simulink model "Test1_2"  (R2021a)
settings: Solver=FixedStepAuto  StartTime=0  StopTime=0.2  FixedStep=0.2  RelTol=1e-3
libraries: spsDistributedParametersLineLib x60, spsThreePhaseSeriesRLCLoadLib x20, spsThreePhaseVIMeasurementLib x4, spsGroundLib x1, spsThreePhaseSourceLib x1, spsSeriesRLCBranchLib x1, spspowerguiLib x1
settings Model: Creator=Admin  LastModifiedBy=Admin

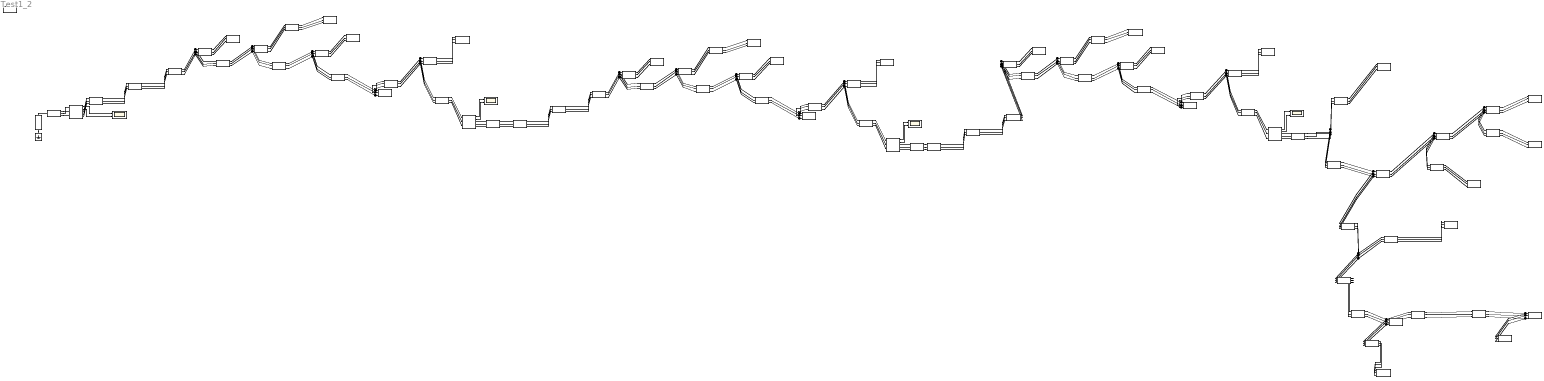
== system Test1_2 ==
  Ground : spsGroundLib/Ground  LConnTagsString=a
  Line 1 : spsDistributedParametersLineLib/Distributed Parameters Line  Phases=3  Length=0.24  Frequency=50  Resistance=[0.646656091154803 0.0486237908083191 0.0486712220507153;0.0486237908083191 0.646561225344642 0.0486237934466192;0.0486712220507153 0.0486237934466192 0.646656091154803]  Inductance=[0.00282448912315926 0.00133270803418135 0.00132951476746136;0.00133270803418135 0.00282479813276775 0.00133799988507366;0.00132951476746136 0.00133799988507366 0.00282448912315926]  Capacitance=[7.89543174552926e-09 -1.85986777702161e-09 -1.7901190036642e-09;-1.85986777702161e-09 7.82540023894543e-09 -1.8957321828871e-09;-1.7901190036642e-09 -1.8957321828871e-09 7.91264394645417e-09]  x1=[156.965405779652 1871.38054427965 1874.40865599682;314.159265358979 314.159265358979 314.159265358979;0.993745600560131 -0.794119316260784 -2.36332785011813]  x2=[156.969311652178 1871.26228409431 1874.29035744918;314.159265358979 314.159265358979 314.159265358979;0.993735016582748 -0.794173336848075 -2.36338159096693]  x3=[0.137596682921067 3.90971974679108 3.95295362832676;314.159265358979 314.159265358979 314.159265358979;0.924963946831068 -0.803256789057363 -2.37264678467375]  x4=[0.137502761428777 5.61255406681359 5.65797563637533;314.159265358979 314.159265358979 314.159265358979;1.0622023156878 -0.788043484537009 -2.35710686392184]  x5=1.14995345102668e-06  V1=ones(3,3)  V2=ones(3,3)  I1=ones(3,3)  I2=ones(3,3)  nHarmo=1  Measurements=None  Decoupling=off  VsMag0=0  VrMag0=0  VsAngle0=0  VrAngle0=0  IsMag0=0  IrMag0=0  IsAngle0=0  IrAngle0=0
      settings: SourceProductBaseCode=PS
  Line 10 : spsDistributedParametersLineLib/Distributed Parameters Line  Phases=3  Length=0.17001  Frequency=50  Resistance=[0.646656091154803 0.0486237908083191 0.0486712220507153;0.0486237908083191 0.646561225344642 0.0486237934466192;0.0486712220507153 0.0486237934466192 0.646656091154803]  Inductance=[0.00282448912315926 0.00133270803418135 0.00132951476746136;0.00133270803418135 0.00282479813276775 0.00133799988507366;0.00132951476746136 0.00133799988507366 0.00282448912315926]  Capacitance=[7.89543174552926e-09 -1.85986777702161e-09 -1.7901190036642e-09;-1.85986777702161e-09 7.82540023894543e-09 -1.8957321828871e-09;-1.7901190036642e-09 -1.8957321828871e-09 7.91264394645417e-09]  x1=[152.36017586446 2437.89117531741 2440.98179824564;314.159265358979 314.159265358979 314.159265358979;0.986975522658831 -0.641771871808401 -2.211874437678]  x2=[152.360654227211 2437.82903835373 2440.91967974814;314.159265358979 314.159265358979 314.159265358979;0.986975936673677 -0.641781263273401 -2.21188373356873]  x3=[0.133985232494409 5.71786094267282 5.77269147189891;314.159265358979 314.159265358979 314.159265358979;0.97714846741076 -0.614289076815549 -2.18464823198113]  x4=[0.132433471923299 6.69193998518046 6.74818842330152;314.159265358979 314.159265358979 314.159265358979;0.996660724368349 -0.66545069261843 -2.23536155506213]  x5=8.14598275871021e-07  V1=ones(3,3)  V2=ones(3,3)  I1=ones(3,3)  I2=ones(3,3)  nHarmo=1  Measurements=None  Decoupling=off  VsMag0=0  VrMag0=0  VsAngle0=0  VrAngle0=0  IsMag0=0  IrMag0=0  IsAngle0=0  IrAngle0=0
      settings: SourceProductBaseCode=PS
  Line 11 : spsDistributedParametersLineLib/Distributed Parameters Line  Phases=3  Length=0.27999  Frequency=50  Resistance=[0.646656091154803 0.0486237908083191 0.0486712220507153;0.0486237908083191 0.646561225344642 0.0486237934466192;0.0486712220507153 0.0486237934466192 0.646656091154803]  Inductance=[0.00282448912315926 0.00133270803418135 0.00132951476746136;0.00133270803418135 0.00282479813276775 0.00133799988507366;0.00132951476746136 0.00133799988507366 0.00282448912315926]  Capacitance=[7.89543174552926e-09 -1.85986777702161e-09 -1.7901190036642e-09;-1.85986777702161e-09 7.82540023894543e-09 -1.8957321828871e-09;-1.7901190036642e-09 -1.8957321828871e-09 7.91264394645417e-09]  x1=[149.797050896305 2771.33912653979 2774.29965117019;314.159265358979 314.159265358979 314.159265358979;0.982741259196518 -0.584603477585544 -2.15500920101434]  x2=[152.36017586446 2437.89117531741 2440.98179824564;314.159265358979 314.159265358979 314.159265358979;0.98680997135433 -0.641903391446747 -2.21200608251373]  x3=[5.10032716906624 1708.06752482602 1710.82869814989;314.159265358979 314.159265358979 314.159265358979;0.0770321916931183 2.28203627723541 0.713549765238094]  x4=[4.94208106497761 1720.91266597234 1723.79335570085;314.159265358979 314.159265358979 314.159265358979;-3.10669073601587 -0.857667050459027 -2.42615340559462]  x5=1.341564444804e-06  V1=ones(3,3)  V2=ones(3,3)  I1=ones(3,3)  I2=ones(3,3)  nHarmo=1  Measurements=None  Decoupling=off  VsMag0=0  VrMag0=0  VsAngle0=0  VrAngle0=0  IsMag0=0  IrMag0=0  IsAngle0=0  IrAngle0=0
      settings: SourceProductBaseCode=PS
  Line 12 : spsDistributedParametersLineLib/Distributed Parameters Line  Phases=3  Length=0.01  Frequency=50  Resistance=[0.646656091154803 0.0486237908083191 0.0486712220507153;0.0486237908083191 0.646561225344642 0.0486237934466192;0.0486712220507153 0.0486237934466192 0.646656091154803]  Inductance=[0.00282448912315926 0.00133270803418135 0.00132951476746136;0.00133270803418135 0.00282479813276775 0.00133799988507366;0.00132951476746136 0.00133799988507366 0.00282448912315926]  Capacitance=[7.89543174552926e-09 -1.85986777702161e-09 -1.7901190036642e-09;-1.85986777702161e-09 7.82540023894543e-09 -1.8957321828871e-09;-1.7901190036642e-09 -1.8957321828871e-09 7.91264394645417e-09]  x1=[149.705553633054 2783.39576802834 2786.35027775329;314.159265358979 314.159265358979 314.159265358979;0.982999779940424 -0.582489121625129 -2.15290363454968]  x2=[149.797050896305 2771.33912653979 2774.29965117019;314.159265358979 314.159265358979 314.159265358979;0.983147671241456 -0.584280609908175 -2.15468602598981]  x3=[5.10074508935649 1708.39159422601 1711.15572048992;314.159265358979 314.159265358979 314.159265358979;0.0774245703226859 2.28234705420157 0.713860837153466]  x4=[4.94342316518712 1721.99747040041 1724.88811393859;314.159265358979 314.159265358979 314.159265358979;-3.10585986858964 -0.857009678007319 -2.42549540948617]  x5=4.79147271261115e-08  V1=ones(3,3)  V2=ones(3,3)  I1=ones(3,3)  I2=ones(3,3)  nHarmo=1  Measurements=None  Decoupling=off  VsMag0=0  VrMag0=0  VsAngle0=0  VrAngle0=0  IsMag0=0  IrMag0=0  IsAngle0=0  IrAngle0=0
      settings: SourceProductBaseCode=PS
  Line 13 : spsDistributedParametersLineLib/Distributed Parameters Line  Phases=3  Length=0.04  Frequency=50  Resistance=[0.646656091154803 0.0486237908083191 0.0486712220507153;0.0486237908083191 0.646561225344642 0.0486237934466192;0.0486712220507153 0.0486237934466192 0.646656091154803]  Inductance=[0.00282448912315926 0.00133270803418135 0.00132951476746136;0.00133270803418135 0.00282479813276775 0.00133799988507366;0.00132951476746136 0.00133799988507366 0.00282448912315926]  Capacitance=[7.89543174552926e-09 -1.85986777702161e-09 -1.7901190036642e-09;-1.85986777702161e-09 7.82540023894543e-09 -1.8957321828871e-09;-1.7901190036642e-09 -1.8957321828871e-09 7.91264394645417e-09]  x1=[149.339597083059 2831.70975798566 2834.63941721022;314.159265358979 314.159265358979 314.159265358979;0.982361245048393 -0.575511762998782 -2.14596168775407]  x2=[149.705553633055 2783.39576802834 2786.35027775329;314.159265358979 314.159265358979 314.159265358979;0.982954621374002 -0.582524997140226 -2.15293954421573]  x3=[5.10056470112681 1708.24829976189 1711.01111492172;314.159265358979 314.159265358979 314.159265358979;0.0773196242206305 2.28226328792446 0.713776990731191]  x4=[4.94340800824378 1721.98418896766 1724.87470903959;314.159265358979 314.159265358979 314.159265358979;-3.10588973167749 -0.857033624646841 -2.42551937913716]  x5=1.91658908504446e-07  V1=ones(3,3)  V2=ones(3,3)  I1=ones(3,3)  I2=ones(3,3)  nHarmo=1  Measurements=None  Decoupling=off  VsMag0=0  VrMag0=0  VsAngle0=0  VrAngle0=0  IsMag0=0  IrMag0=0  IsAngle0=0  IrAngle0=0
      settings: SourceProductBaseCode=PS
  Line 14 : spsDistributedParametersLineLib/Distributed Parameters Line  Phases=3  Length=0.24001  Frequency=50  Resistance=[0.646656091154803 0.0486237908083191 0.0486712220507153;0.0486237908083191 0.646561225344642 0.0486237934466192;0.0486712220507153 0.0486237934466192 0.646656091154803]  Inductance=[0.00282448912315926 0.00133270803418135 0.00132951476746136;0.00133270803418135 0.00282479813276775 0.00133799988507366;0.00132951476746136 0.00133799988507366 0.00282448912315926]  Capacitance=[7.89543174552926e-09 -1.85986777702161e-09 -1.7901190036642e-09;-1.85986777702161e-09 7.82540023894543e-09 -1.8957321828871e-09;-1.7901190036642e-09 -1.8957321828871e-09 7.91264394645417e-09]  x1=[147.366559624798 3124.27831554393 3127.12738116645;314.159265358979 314.159265358979 314.159265358979;0.977740300651082 -0.53827513849313 -2.10890856037845]  x2=[149.339597082437 2831.70975810682 2834.63941733118;314.159265358979 314.159265358979 314.159265358979;0.982060172883721 -0.575750945040668 -2.14620109748057]  x3=[4.69597972482398 1707.56618859991 1710.7915439131;314.159265358979 314.159265358979 314.159265358979;0.150881701422709 2.28144587423602 0.712853079667161]  x4=[4.52474633855033 1722.028392532 1725.38783678718;314.159265358979 314.159265358979 314.159265358979;-3.03298242084286 -0.857513917481596 -2.42610561272272]  x5=1.1500013657538e-06  V1=ones(3,3)  V2=ones(3,3)  I1=ones(3,3)  I2=ones(3,3)  nHarmo=1  Measurements=None  Decoupling=off  VsMag0=0  VrMag0=0  VsAngle0=0  VrAngle0=0  IsMag0=0  IrMag0=0  IsAngle0=0  IrAngle0=0
      settings: SourceProductBaseCode=PS
  Line 15 : spsDistributedParametersLineLib/Distributed Parameters Line  Phases=3  Length=0.17  Frequency=50  Resistance=[0.646656091154803 0.0486237908083191 0.0486712220507153;0.0486237908083191 0.646561225344642 0.0486237934466192;0.0486712220507153 0.0486237934466192 0.646656091154803]  Inductance=[0.00282448912315926 0.00133270803418135 0.00132951476746136;0.00133270803418135 0.00282479813276775 0.00133799988507366;0.00132951476746136 0.00133799988507366 0.00282448912315926]  Capacitance=[7.89543174552926e-09 -1.85986777702161e-09 -1.7901190036642e-09;-1.85986777702161e-09 7.82540023894543e-09 -1.8957321828871e-09;-1.7901190036642e-09 -1.8957321828871e-09 7.91264394645417e-09]  x1=[132.899841984529 5355.36116411885 5357.02335058589;314.159265358979 314.159265358979 314.159265358979;0.942020039880082 -0.391447182887755 -1.96269694426104]  x2=[132.900799709299 5355.22518061845 5356.8875370799;314.159265358979 314.159265358979 314.159265358979;0.942023005810223 -0.391455476704388 -1.96270514529814]  x3=[0.118536716166914 12.5926352479183 12.7008603036067;314.159265358979 314.159265358979 314.159265358979;0.922749204209291 -0.36138822130875 -1.93290685330754]  x4=[0.113887175748437 14.6699901164864 14.7794661915918;314.159265358979 314.159265358979 314.159265358979;0.961819622301432 -0.417445208664834 -1.98849312716543]  x5=8.14550361143895e-07  V1=ones(3,3)  V2=ones(3,3)  I1=ones(3,3)  I2=ones(3,3)  nHarmo=1  Measurements=None  Decoupling=off  VsMag0=0  VrMag0=0  VsAngle0=0  VrAngle0=0  IsMag0=0  IrMag0=0  IsAngle0=0  IrAngle0=0
      settings: SourceProductBaseCode=PS
  Line 16 : spsDistributedParametersLineLib/Distributed Parameters Line  Phases=3  Length=0.27999  Frequency=50  Resistance=[0.646656091154803 0.0486237908083191 0.0486712220507153;0.0486237908083191 0.646561225344642 0.0486237934466192;0.0486712220507153 0.0486237934466192 0.646656091154803]  Inductance=[0.00282448912315926 0.00133270803418135 0.00132951476746136;0.00133270803418135 0.00282479813276775 0.00133799988507366;0.00132951476746136 0.00133799988507366 0.00282448912315926]  Capacitance=[7.89543174552926e-09 -1.85986777702161e-09 -1.7901190036642e-09;-1.85986777702161e-09 7.82540023894543e-09 -1.8957321828871e-09;-1.7901190036642e-09 -1.8957321828871e-09 7.91264394645417e-09]  x1=[130.625805916313 5714.43330932926 5715.86450257811;314.159265358979 314.159265358979 314.159265358979;0.935455723402759 -0.378911532038673 -1.9502060628031]  x2=[132.899841984529 5355.36116411885 5357.02335058588;314.159265358979 314.159265358979 314.159265358979;0.941854473522726 -0.391578714484606 -1.96282860106665]  x3=[4.69943627260133 1705.04689657621 1708.22372245339;314.159265358979 314.159265358979 314.159265358979;0.147579410474112 2.27912018503212 0.710521164983193]  x4=[4.54038793511918 1730.11014591192 1733.52103743161;314.159265358979 314.159265358979 314.159265358979;-3.03009591800017 -0.854995304416789 -2.42358856047792]  x5=1.341564444804e-06  V1=ones(3,3)  V2=ones(3,3)  I1=ones(3,3)  I2=ones(3,3)  nHarmo=1  Measurements=None  Decoupling=off  VsMag0=0  VrMag0=0  VsAngle0=0  VrAngle0=0  IsMag0=0  IrMag0=0  IsAngle0=0  IrAngle0=0
      settings: SourceProductBaseCode=PS
  Line 17 : spsDistributedParametersLineLib/Distributed Parameters Line  Phases=3  Length=0.01  Frequency=50  Resistance=[0.646656091154803 0.0486237908083191 0.0486712220507153;0.0486237908083191 0.646561225344642 0.0486237934466192;0.0486712220507153 0.0486237934466192 0.646656091154803]  Inductance=[0.00282448912315926 0.00133270803418135 0.00132951476746136;0.00133270803418135 0.00282479813276775 0.00133799988507366;0.00132951476746136 0.00133799988507366 0.00282448912315926]  Capacitance=[7.89543174552926e-09 -1.85986777702161e-09 -1.7901190036642e-09;-1.85986777702161e-09 7.82540023894543e-09 -1.8957321828871e-09;-1.7901190036642e-09 -1.8957321828871e-09 7.91264394645417e-09]  x1=[130.544687715025 5727.27361859197 5728.69645510391;314.159265358979 314.159265358979 314.159265358979;0.935629480507103 -0.378165636098579 -1.9494613242192]  x2=[130.625805916313 5714.43330932926 5715.86450257811;314.159265358979 314.159265358979 314.159265358979;0.935862135447697 -0.378588664361305 -1.94988288777856]  x3=[4.69982164193658 1705.36967379669 1708.54951574632;314.159265358979 314.159265358979 314.159265358979;0.147971637319338 2.2794306267218 0.710831898749288]  x4=[4.5416219595263 1731.19877594442 1734.619968649;314.159265358979 314.159265358979 314.159265358979;-3.0292654752636 -0.854338819679799 -2.42293145950432]  x5=4.79147271261115e-08  V1=ones(3,3)  V2=ones(3,3)  I1=ones(3,3)  I2=ones(3,3)  nHarmo=1  Measurements=None  Decoupling=off  VsMag0=0  VrMag0=0  VsAngle0=0  VrAngle0=0  IsMag0=0  IrMag0=0  IsAngle0=0  IrAngle0=0
      settings: SourceProductBaseCode=PS
  Line 18 : spsDistributedParametersLineLib/Distributed Parameters Line  Phases=3  Length=0.04  Frequency=50  Resistance=[0.646656091154803 0.0486237908083191 0.0486712220507153;0.0486237908083191 0.646561225344642 0.0486237934466192;0.0486712220507153 0.0486237934466192 0.646656091154803]  Inductance=[0.00282448912315926 0.00133270803418135 0.00132951476746136;0.00133270803418135 0.00282479813276775 0.00133799988507366;0.00132951476746136 0.00133799988507366 0.00282448912315926]  Capacitance=[7.89543174552926e-09 -1.85986777702161e-09 -1.7901190036642e-09;-1.85986777702161e-09 7.82540023894543e-09 -1.8957321828871e-09;-1.7901190036642e-09 -1.8957321828871e-09 7.91264394645417e-09]  x1=[130.220285493845 5778.64498268911 5780.03432477456;314.159265358979 314.159265358979 314.159265358979;0.934650804974626 -0.376528198600221 -1.94782969786199]  x2=[130.544687715024 5727.27361859198 5728.69645510391;314.159265358979 314.159265358979 314.159265358979;0.935584321940681 -0.378201511613676 -1.94949723388525]  x3=[4.69965556978429 1705.22633120538 1708.40482377799;314.159265358979 314.159265358979 314.159265358979;0.1478666288771 2.27934671978969 0.710747910420055]  x4=[4.54160812738084 1731.18526113571 1734.60632300578;314.159265358979 314.159265358979 314.159265358979;-3.02929537261956 -0.854362839392123 -2.4229555028762]  x5=1.91658908504446e-07  V1=ones(3,3)  V2=ones(3,3)  I1=ones(3,3)  I2=ones(3,3)  nHarmo=1  Measurements=None  Decoupling=off  VsMag0=0  VrMag0=0  VsAngle0=0  VrAngle0=0  IsMag0=0  IrMag0=0  IsAngle0=0  IrAngle0=0
      settings: SourceProductBaseCode=PS
  Line 19 : spsDistributedParametersLineLib/Distributed Parameters Line  Phases=3  Length=0.02  Frequency=50  Resistance=[0.646656091154803 0.0486237908083191 0.0486712220507153;0.0486237908083191 0.646561225344642 0.0486237934466192;0.0486712220507153 0.0486237934466192 0.646656091154803]  Inductance=[0.00282448912315926 0.00133270803418135 0.00132951476746136;0.00133270803418135 0.00282479813276775 0.00133799988507366;0.00132951476746136 0.00133799988507366 0.00282448912315926]  Capacitance=[7.89543174552926e-09 -1.85986777702161e-09 -1.7901190036642e-09;-1.85986777702161e-09 7.82540023894543e-09 -1.8957321828871e-09;-1.7901190036642e-09 -1.8957321828871e-09 7.91264394645417e-09]  x1=[147.366559624798 3124.27831554393 3127.12738116645;314.159265358979 314.159265358979 314.159265358979;0.978071478524361 -0.538012039423913 -2.10864521085755]  x2=[147.366576589391 3124.27609299989 3127.1251586601;314.159265358979 314.159265358979 314.159265358979;0.978071529284701 -0.538012448077892 -2.10864561647098]  x3=[0.129209254301903 7.78403106502851 7.85222208431091;314.159265358979 314.159265358979 314.159265358979;0.975452703470751 -0.534902174377798 -2.10556665489213]  x4=[0.128484600405194 8.11756536104211 8.18611566687072;314.159265358979 314.159265358979 314.159265358979;0.980674883603026 -0.5410179521277 -2.11162204802365]  x5=9.5829454252223e-08  V1=ones(3,3)  V2=ones(3,3)  I1=ones(3,3)  I2=ones(3,3)  nHarmo=1  Measurements=None  Decoupling=off  VsMag0=0  VrMag0=0  VsAngle0=0  VrAngle0=0  IsMag0=0  IrMag0=0  IsAngle0=0  IrAngle0=0
      settings: SourceProductBaseCode=PS
  Line 2 : spsDistributedParametersLineLib/Distributed Parameters Line  Phases=3  Length=0.02  Frequency=50  Resistance=[0.646656091154803 0.0486237908083191 0.0486712220507153;0.0486237908083191 0.646561225344642 0.0486237934466192;0.0486712220507153 0.0486237934466192 0.646656091154803]  Inductance=[0.00282448912315926 0.00133270803418135 0.00132951476746136;0.00133270803418135 0.00282479813276775 0.00133799988507366;0.00132951476746136 0.00133799988507366 0.00282448912315926]  Capacitance=[7.89543174552926e-09 -1.85986777702161e-09 -1.7901190036642e-09;-1.85986777702161e-09 7.82540023894543e-09 -1.8957321828871e-09;-1.7901190036642e-09 -1.8957321828871e-09 7.91264394645417e-09]  x1=[156.965405779652 1871.38054427965 1874.40865599682;314.159265358979 314.159265358979 314.159265358979;0.994076763380555 -0.793856229150073 -2.36306451256712]  x2=[156.965417517027 1871.37888626964 1874.40699915953;314.159265358979 314.159265358979 314.159265358979;0.994076744009357 -0.793856337139222 -2.3630646177889]  x3=[0.137288875738453 4.66877336660217 4.71294070353627;314.159265358979 314.159265358979 314.159265358979;0.991734266986629 -0.781676589050808 -2.3509868412552]  x4=[0.137189890045939 4.85660166120808 4.9011132957881;314.159265358979 314.159265358979 314.159265358979;0.996390813875115 -0.805588362177722 -2.3747020378792]  x5=9.5829454252223e-08  V1=ones(3,3)  V2=ones(3,3)  I1=ones(3,3)  I2=ones(3,3)  nHarmo=1  Measurements=None  Decoupling=off  VsMag0=0  VrMag0=0  VsAngle0=0  VrAngle0=0  IsMag0=0  IrMag0=0  IsAngle0=0  IrAngle0=0
      settings: SourceProductBaseCode=PS
  Line 20 : spsDistributedParametersLineLib/Distributed Parameters Line  Phases=3  Length=0.5  Frequency=50  Resistance=[0.646656091154803 0.0486237908083191 0.0486712220507153;0.0486237908083191 0.646561225344642 0.0486237934466192;0.0486712220507153 0.0486237934466192 0.646656091154803]  Inductance=[0.00282448912315926 0.00133270803418135 0.00132951476746136;0.00133270803418135 0.00282479813276775 0.00133799988507366;0.00132951476746136 0.00133799988507366 0.00282448912315926]  Capacitance=[7.89543174552926e-09 -1.85986777702161e-09 -1.7901190036642e-09;-1.85986777702161e-09 7.82540023894543e-09 -1.8957321828871e-09;-1.7901190036642e-09 -1.8957321828871e-09 7.91264394645417e-09]  x1=[143.264957244536 3744.49816369777 3747.08832907544;314.159265358979 314.159265358979 314.159265358979;0.967966773621725 -0.479516643242202 -2.05041928603723]  x2=[147.366559624798 3124.27831554393 3127.12738116645;314.159265358979 314.159265358979 314.159265358979;0.977348941461618 -0.538586047665466 -2.1092197655143]  x3=[4.69457824125427 1706.09065502595 1709.30076063797;314.159265358979 314.159265358979 314.159265358979;0.149751318444868 2.28055339272289 0.71195954517954]  x4=[4.52557826260862 1722.47910674114 1725.84144140248;314.159265358979 314.159265358979 314.159265358979;-3.03299533225323 -0.85752144723027 -2.42611334880867]  x5=2.39573635630557e-06  V1=ones(3,3)  V2=ones(3,3)  I1=ones(3,3)  I2=ones(3,3)  nHarmo=1  Measurements=None  Decoupling=off  VsMag0=0  VrMag0=0  VsAngle0=0  VrAngle0=0  IsMag0=0  IrMag0=0  IsAngle0=0  IrAngle0=0
      settings: SourceProductBaseCode=PS
  Line 21 : spsDistributedParametersLineLib/Distributed Parameters Line  Phases=3  Length=0.23  Frequency=50  Resistance=[0.646656091154803 0.0486237908083191 0.0486712220507153;0.0486237908083191 0.646561225344642 0.0486237934466192;0.0486712220507153 0.0486237934466192 0.646656091154803]  Inductance=[0.00282448912315926 0.00133270803418135 0.00132951476746136;0.00133270803418135 0.00282479813276775 0.00133799988507366;0.00132951476746136 0.00133799988507366 0.00282448912315926]  Capacitance=[7.89543174552926e-09 -1.85986777702161e-09 -1.7901190036642e-09;-1.85986777702161e-09 7.82540023894543e-09 -1.8957321828871e-09;-1.7901190036642e-09 -1.8957321828871e-09 7.91264394645417e-09]  x1=[141.381540716079 4033.34520134928 4035.78863035435;314.159265358979 314.159265358979 314.159265358979;0.963872150999868 -0.458142281050839 -2.02913402389008]  x2=[143.264957244536 3744.49816369777 3747.08832907544;314.159265358979 314.159265358979 314.159265358979;0.968373200719517 -0.479193763606329 -2.05009609904281]  x3=[4.69693280636161 1706.73403429122 1709.94265597579;314.159265358979 314.159265358979 314.159265358979;0.149813372942936 2.28064855389235 0.712053657755716]  x4=[4.53009342094595 1725.03316244308 1728.41207132862;314.159265358979 314.159265358979 314.159265358979;-3.03180886302381 -0.856556207454851 -2.42514832021994]  x5=1.10203872390056e-06  V1=ones(3,3)  V2=ones(3,3)  I1=ones(3,3)  I2=ones(3,3)  nHarmo=1  Measurements=None  Decoupling=off  VsMag0=0  VrMag0=0  VsAngle0=0  VrAngle0=0  IsMag0=0  IrMag0=0  IsAngle0=0  IrAngle0=0
      settings: SourceProductBaseCode=PS
  Line 22 : spsDistributedParametersLineLib/Distributed Parameters Line  Phases=3  Length=1.62  Frequency=50  Resistance=[0.80718830189013 0.0486237908083191 0.0486712220507153;0.0486237908083191 0.807093436079969 0.0486237934466192;0.0486712220507153 0.0486237934466192 0.80718830189013]  Inductance=[0.00279786707424938 0.00133270803418135 0.00132951476746136;0.00133270803418135 0.00279817608385787 0.00133799988507366;0.00132951476746136 0.00133799988507366 0.00279786707424938]  Capacitance=[7.73340098830622e-09 -1.79942827973291e-09 -1.73218055098733e-09;-1.79942827973291e-09 7.66505189233746e-09 -1.83375898618858e-09;-1.73218055098733e-09 -1.83375898618858e-09 7.749673531177e-09]  x1=[111.255817895821 4033.38117611576 4036.11238880674;314.159265358979 314.159265358979 314.159265358979;1.03593595279213 -0.464052863724388 -2.03502879066849]  x2=[111.256284671676 4033.37738573713 4036.10862101927;314.159265358979 314.159265358979 314.159265358979;1.03593486115945 -0.464056537743729 -2.03503248077632]  x3=[0.0968983486960544 10.2070175470074 10.2916609188853;314.159265358979 314.159265358979 314.159265358979;1.03318306869383 -0.465730267618516 -2.03670968562963]  x4=[0.0968282868719981 10.2221861600155 10.3068418342109;314.159265358979 314.159265358979 314.159265358979;1.03626767416038 -0.464279740581859 -2.03525380445823]  x5=7.70442045759223e-06  V1=ones(3,3)  V2=ones(3,3)  I1=ones(3,3)  I2=ones(3,3)  nHarmo=1  Measurements=None  Decoupling=off  VsMag0=0  VrMag0=0  VsAngle0=0  VrAngle0=0  IsMag0=0  IrMag0=0  IsAngle0=0  IrAngle0=0
      settings: SourceProductBaseCode=PS
  Line 23 : spsDistributedParametersLineLib/Distributed Parameters Line  Phases=3  Length=0.54002  Frequency=50  Resistance=[0.646656091154803 0.0486237908083191 0.0486712220507153;0.0486237908083191 0.646561225344642 0.0486237934466192;0.0486712220507153 0.0486237934466192 0.646656091154803]  Inductance=[0.00282448912315926 0.00133270803418135 0.00132951476746136;0.00133270803418135 0.00282479813276775 0.00133799988507366;0.00132951476746136 0.00133799988507366 0.00282448912315926]  Capacitance=[7.89543174552926e-09 -1.85986777702161e-09 -1.7901190036642e-09;-1.85986777702161e-09 7.82540023894543e-09 -1.8957321828871e-09;-1.7901190036642e-09 -1.8957321828871e-09 7.91264394645417e-09]  x1=[136.970854809158 4717.10989026672 4719.16622621704;314.159265358979 314.159265358979 314.159265358979;0.952352588146702 -0.419268144212771 -1.99041696083254]  x2=[141.381540716079 4033.34520134928 4035.78863035435;314.159265358979 314.159265358979 314.159265358979;0.963405482374469 -0.458513018623851 -2.02950511437901]  x3=[4.6950771769482 1704.92349425677 1708.11503821512;314.159265358979 314.159265358979 314.159265358979;0.1484970320043 2.2796412280549 0.711045424706869]  x4=[4.53057574604281 1725.22598750204 1728.60666973103;314.159265358979 314.159265358979 314.159265358979;-3.03196710314176 -0.856642086949454 -2.42523422570912]  x5=2.58749109426427e-06  V1=ones(3,3)  V2=ones(3,3)  I1=ones(3,3)  I2=ones(3,3)  nHarmo=1  Measurements=None  Decoupling=off  VsMag0=0  VrMag0=0  VsAngle0=0  VrAngle0=0  IsMag0=0  IrMag0=0  IsAngle0=0  IrAngle0=0
      settings: SourceProductBaseCode=PS
  Line 24 : spsDistributedParametersLineLib/Distributed Parameters Line  Phases=3  Length=0.13998  Frequency=50  Resistance=[0.646656091154803 0.0486237908083191 0.0486712220507153;0.0486237908083191 0.646561225344642 0.0486237934466192;0.0486712220507153 0.0486237934466192 0.646656091154803]  Inductance=[0.00282448912315926 0.00133270803418135 0.00132951476746136;0.00133270803418135 0.00282479813276775 0.00133799988507366;0.00132951476746136 0.00133799988507366 0.00282448912315926]  Capacitance=[7.89543174552926e-09 -1.85986777702161e-09 -1.7901190036642e-09;-1.85986777702161e-09 7.82540023894543e-09 -1.8957321828871e-09;-1.7901190036642e-09 -1.8957321828871e-09 7.91264394645417e-09]  x1=[136.970854809158 4717.10989026672 4719.16622621704;314.159265358979 314.159265358979 314.159265358979;0.952954762577076 -0.418789756177456 -1.98993811740569]  x2=[136.971666154249 4717.03540311946 4719.09183073719;314.159265358979 314.159265358979 314.159265358979;0.952955500131483 -0.418794373833103 -1.98994267847764]  x3=[0.121357845438818 11.3292840292329 11.4262147740208;314.159265358979 314.159265358979 314.159265358979;0.930714707543745 -0.394910744474516 -1.96626658224448]  x4=[0.118203608434895 12.6819047773621 12.7798105880992;314.159265358979 314.159265358979 314.159265358979;0.975575610247598 -0.440284325346567 -2.01126504900171]  x5=6.70710350311308e-07  V1=ones(3,3)  V2=ones(3,3)  I1=ones(3,3)  I2=ones(3,3)  nHarmo=1  Measurements=None  Decoupling=off  VsMag0=0  VrMag0=0  VsAngle0=0  VrAngle0=0  IsMag0=0  IrMag0=0  IsAngle0=0  IrAngle0=0
      settings: SourceProductBaseCode=PS
  Line 25 : spsDistributedParametersLineLib/Distributed Parameters Line  Phases=3  Length=0.14997  Frequency=50  Resistance=[0.476003738225748 0.351747138225748 0.351747138225748;0.351747138225748 0.476003738225748 0.351747138225748;0.351747138225748 0.351747138225748 0.476003738225748]  Inductance=[0.000705954362986426 0.000459934243504405 0.000459934243504405;0.000459934243504405 0.000705954362986426 0.000459934243504405;0.000459934243504405 0.000459934243504405 0.000705954362986426]  Capacitance=[5.7561313269996e-07 -1.37543883484145e-07 -1.37543912800485e-07;-1.37543883484145e-07 5.75613027339387e-07 -1.37543875208088e-07;-1.37543912800485e-07 -1.37543875208088e-07 5.75613005057695e-07]  x1=[77.3212987177548 4717.59725972927 4719.75403690061;314.159265358979 314.159265358979 314.159265358979;1.09142381613903 -0.337596063619059 -1.90863201691887]  x2=[77.3213406496756 4717.58057530735 4719.73734485071;314.159265358979 314.159265358979 314.159265358979;1.09142256389172 -0.337596336996628 -1.90863229029648]  x3=[1.04934913172663 253.129562662736 253.245268059759;314.159265358979 314.159265358979 314.159265358979;1.09038177152188 -0.336520492000803 -1.9075564451716]  x4=[1.04934910448407 254.481417052228 254.59774051285;314.159265358979 314.159265358979 314.159265358979;1.09142254929381 -0.339288761111601 -1.91032471449075]  x5=3.31498451375949e-06  V1=ones(3,3)  V2=ones(3,3)  I1=ones(3,3)  I2=ones(3,3)  nHarmo=1  Measurements=None  Decoupling=off  VsMag0=0  VrMag0=0  VsAngle0=0  VrAngle0=0  IsMag0=0  IrMag0=0  IsAngle0=0  IrAngle0=0
      settings: SourceProductBaseCode=PS
  Line 26 : spsDistributedParametersLineLib/Distributed Parameters Line  Phases=3  Length=0.50001  Frequency=50  Resistance=[0.646656091154803 0.0486237908083191 0.0486712220507153;0.0486237908083191 0.646561225344642 0.0486237934466192;0.0486712220507153 0.0486237934466192 0.646656091154803]  Inductance=[0.00282448912315926 0.00133270803418135 0.00132951476746136;0.00133270803418135 0.00282479813276775 0.00133799988507366;0.00132951476746136 0.00133799988507366 0.00282448912315926]  Capacitance=[7.89543174552926e-09 -1.85986777702161e-09 -1.7901190036642e-09;-1.85986777702161e-09 7.82540023894543e-09 -1.8957321828871e-09;-1.7901190036642e-09 -1.8957321828871e-09 7.91264394645417e-09]  x1=[132.899841984529 5355.36116411885 5357.02335058589;314.159265358979 314.159265358979 314.159265358979;0.941523280596591 -0.391841825512328 -1.96309196255744]  x2=[136.970854809158 4717.10989026672 4719.16622621704;314.159265358979 314.159265358979 314.159265358979;0.952412814621452 -0.419220298234136 -1.99036906930793]  x3=[4.69667848159883 1704.39660768418 1707.57684651848;314.159265358979 314.159265358979 314.159265358979;0.147653797922356 2.27911528105476 0.710517948064024]  x4=[4.53531416160052 1727.41542933722 1730.81042696937;314.159265358979 314.159265358979 314.159265358979;-3.0312239923196 -0.855926939645363 -2.42451941049668]  x5=2.3957842710327e-06  V1=ones(3,3)  V2=ones(3,3)  I1=ones(3,3)  I2=ones(3,3)  nHarmo=1  Measurements=None  Decoupling=off  VsMag0=0  VrMag0=0  VsAngle0=0  VrAngle0=0  IsMag0=0  IrMag0=0  IsAngle0=0  IrAngle0=0
      settings: SourceProductBaseCode=PS
  Line 3 : spsDistributedParametersLineLib/Distributed Parameters Line  Phases=3  Length=0.5  Frequency=50  Resistance=[0.646656091154803 0.0486237908083191 0.0486712220507153;0.0486237908083191 0.646561225344642 0.0486237934466192;0.0486712220507153 0.0486237934466192 0.646656091154803]  Inductance=[0.00282448912315926 0.00133270803418135 0.00132951476746136;0.00133270803418135 0.00282479813276775 0.00133799988507366;0.00132951476746136 0.00133799988507366 0.00282448912315926]  Capacitance=[7.89543174552926e-09 -1.85986777702161e-09 -1.7901190036642e-09;-1.85986777702161e-09 7.82540023894543e-09 -1.8957321828871e-09;-1.7901190036642e-09 -1.8957321828871e-09 7.91264394645417e-09]  x1=[156.956907595247 1871.66787959428 1874.69603995596;314.159265358979 314.159265358979 314.159265358979;0.993376948009191 -0.794314673924448 -2.36352415263414]  x2=[156.965405779652 1871.38054427965 1874.40865599682;314.159265358979 314.159265358979 314.159265358979;0.993354226317812 -0.794430237391626 -2.36363906722387]  x3=[0.137650868781888 3.81520206109773 3.85823350187218;314.159265358979 314.159265358979 314.159265358979;0.92153433973683 -0.789495270500456 -2.35903959755234]  x4=[0.137458609404139 5.70509774441842 5.7506581745733;314.159265358979 314.159265358979 314.159265358979;1.06454424282906 -0.798132971601806 -2.36712903812269]  x5=2.39573635630557e-06  V1=ones(3,3)  V2=ones(3,3)  I1=ones(3,3)  I2=ones(3,3)  nHarmo=1  Measurements=None  Decoupling=off  VsMag0=0  VrMag0=0  VsAngle0=0  VrAngle0=0  IsMag0=0  IrMag0=0  IsAngle0=0  IrAngle0=0
      settings: SourceProductBaseCode=PS
  Line 4 : spsDistributedParametersLineLib/Distributed Parameters Line  Phases=3  Length=0.23  Frequency=50  Resistance=[0.646656091154803 0.0486237908083191 0.0486712220507153;0.0486237908083191 0.646561225344642 0.0486237934466192;0.0486712220507153 0.0486237934466192 0.646656091154803]  Inductance=[0.00282448912315926 0.00133270803418135 0.00132951476746136;0.00133270803418135 0.00282479813276775 0.00133799988507366;0.00132951476746136 0.00133799988507366 0.00282448912315926]  Capacitance=[7.89543174552926e-09 -1.85986777702161e-09 -1.7901190036642e-09;-1.85986777702161e-09 7.82540023894543e-09 -1.8957321828871e-09;-1.7901190036642e-09 -1.8957321828871e-09 7.91264394645417e-09]  x1=[156.952553131653 1871.85294613081 1874.88113522112;314.159265358979 314.159265358979 314.159265358979;0.993793842090127 -0.79392653725406 -2.36313611703891]  x2=[156.956907595247 1871.66787959428 1874.69603995596;314.159265358979 314.159265358979 314.159265358979;0.993783375106984 -0.793991794288575 -2.36320096563972]  x3=[0.138137241015989 3.5006914421516 3.54316106458494;314.159265358979 314.159265358979 314.159265358979;0.915502409980736 -0.764168070499261 -2.33403697280712]  x4=[0.137139558374005 6.02613644564006 6.07225205821398;314.159265358979 314.159265358979 314.159265358979;1.07229801814102 -0.811481059773425 -2.3803832041032]  x5=1.10203872390056e-06  V1=ones(3,3)  V2=ones(3,3)  I1=ones(3,3)  I2=ones(3,3)  nHarmo=1  Measurements=None  Decoupling=off  VsMag0=0  VrMag0=0  VsAngle0=0  VrAngle0=0  IsMag0=0  IrMag0=0  IsAngle0=0  IrAngle0=0
      settings: SourceProductBaseCode=PS
  Line 44 : spsDistributedParametersLineLib/Distributed Parameters Line  Phases=3  Length=1.11  Frequency=50  Resistance=[0.502970710632245 0.0486237908083191 0.0486712220507153;0.0486237908083191 0.502875844822084 0.0486237934466192;0.0486712220507153 0.0486237934466192 0.502970710632245]  Inductance=[0.00286900545038753 0.00133270803418135 0.00132951476746136;0.00133270803418135 0.00286931445999602 0.00133799988507366;0.00132951476746136 0.00133799988507366 0.00286900545038753]  Capacitance=[8.11484299003193e-09 -1.94249816214699e-09 -1.86930692621136e-09;-1.94249816214699e-09 8.0425699231653e-09 -1.98049571960044e-09;-1.86930692621136e-09 -1.98049571960044e-09 8.13337738722527e-09]  x1=[173.362030490119 1870.46864326983 1872.93675817124;314.159265358979 314.159265358979 314.159265358979;0.925429746096986 -0.789510342867653 -2.35873222576214]  x2=[173.362277666248 1870.47039245228 1872.93851360611;314.159265358979 314.159265358979 314.159265358979;0.925429253884466 -0.789511220669717 -2.35873311112546]  x3=[0.151985260585037 4.75806840684685 4.80092870626659;314.159265358979 314.159265358979 314.159265358979;0.923740844335302 -0.790878375878761 -2.36010180165187]  x4=[0.151985260870719 4.75806840784355 4.80092870785854;314.159265358979 314.159265358979 314.159265358979;0.92542925320876 -0.789511220650776 -2.35873311108327]  x5=5.37516004033389e-06  V1=ones(3,3)  V2=ones(3,3)  I1=ones(3,3)  I2=ones(3,3)  nHarmo=1  Measurements=None  Decoupling=off  VsMag0=0  VrMag0=0  VsAngle0=0  VrAngle0=0  IsMag0=0  IrMag0=0  IsAngle0=0  IrAngle0=0
      settings: SourceProductBaseCode=PS
  Line 45 : spsDistributedParametersLineLib/Distributed Parameters Line  Phases=3  Length=0.03  Frequency=50  Resistance=[0.476003738225748 0.351747138225748 0.351747138225748;0.351747138225748 0.476003738225748 0.351747138225748;0.351747138225748 0.351747138225748 0.476003738225748]  Inductance=[0.000705954362986426 0.000459934243504405 0.000459934243504405;0.000459934243504405 0.000705954362986426 0.000459934243504405;0.000459934243504405 0.000459934243504405 0.000705954362986426]  Capacitance=[5.7561313269996e-07 -1.37543883484145e-07 -1.37543912800485e-07;-1.37543883484145e-07 5.75613027339387e-07 -1.37543875208088e-07;-1.37543912800485e-07 -1.37543875208088e-07 5.75613005057695e-07]  x1=[137.574489867811 1870.43821958496 1873.77265383368;314.159265358979 314.159265358979 314.159265358979;1.0926378669217 -0.712734679174021 -2.28197946476194]  x2=[137.574495166611 1870.43824928999 1873.77268368076;314.159265358979 314.159265358979 314.159265358979;1.09263774985956 -0.712734704669924 -2.2819794903938]  x3=[1.86971697622916 100.689759042347 100.869237693452;314.159265358979 314.159265358979 314.159265358979;1.09229955538654 -0.712924192925255 -2.28216957326277]  x4=[1.86979666932282 100.689742781977 100.869248230241;314.159265358979 314.159265358979 314.159265358979;1.09276769806716 -0.712670035796461 -2.28191422679785]  x5=6.63129528657629e-07  V1=ones(3,3)  V2=ones(3,3)  I1=ones(3,3)  I2=ones(3,3)  nHarmo=1  Measurements=None  Decoupling=off  VsMag0=0  VrMag0=0  VsAngle0=0  VrAngle0=0  IsMag0=0  IrMag0=0  IsAngle0=0  IrAngle0=0
      settings: SourceProductBaseCode=PS
  Line 46 : spsDistributedParametersLineLib/Distributed Parameters Line  Phases=3  Length=0.28003  Frequency=50  Resistance=[0.476003738225748 0.351747138225748 0.351747138225748;0.351747138225748 0.476003738225748 0.351747138225748;0.351747138225748 0.351747138225748 0.476003738225748]  Inductance=[0.000705954362986426 0.000459934243504405 0.000459934243504405;0.000459934243504405 0.000705954362986426 0.000459934243504405;0.000459934243504405 0.000459934243504405 0.000705954362986426]  Capacitance=[5.7561313269996e-07 -1.37543883484145e-07 -1.37543912800485e-07;-1.37543883484145e-07 5.75613027339387e-07 -1.37543875208088e-07;-1.37543912800485e-07 -1.37543875208088e-07 5.75613005057695e-07]  x1=[137.574489867811 1870.43821958496 1873.77265383368;314.159265358979 314.159265358979 314.159265358979;1.09090158954707 -0.713775125979268 -2.28301991148676]  x2=[137.574766367975 1870.43959233676 1873.77402962741;314.159265358979 314.159265358979 314.159265358979;1.09089676298152 -0.713776305655424 -2.2830210920491]  x3=[1.86411948827272 100.563600594904 100.74285874572;314.159265358979 314.159265358979 314.159265358979;1.08885867167533 -0.71498806739371 -2.28423327026689]  x4=[1.86417554032863 100.563589510719 100.742865766276;314.159265358979 314.159265358979 314.159265358979;1.0909928599777 -0.713729195375815 -2.2829735644268]  x5=6.18987206366653e-06  V1=ones(3,3)  V2=ones(3,3)  I1=ones(3,3)  I2=ones(3,3)  nHarmo=1  Measurements=None  Decoupling=off  VsMag0=0  VrMag0=0  VsAngle0=0  VrAngle0=0  IsMag0=0  IrMag0=0  IsAngle0=0  IrAngle0=0
      settings: SourceProductBaseCode=PS
  Line 47 : spsDistributedParametersLineLib/Distributed Parameters Line  Phases=3  Length=0.28003  Frequency=50  Resistance=[0.646656091154803 0.0486237908083191 0.0486712220507153;0.0486237908083191 0.646561225344642 0.0486237934466192;0.0486712220507153 0.0486237934466192 0.646656091154803]  Inductance=[0.00282448912315926 0.00133270803418135 0.00132951476746136;0.00133270803418135 0.00282479813276775 0.00133799988507366;0.00132951476746136 0.00133799988507366 0.00282448912315926]  Capacitance=[7.89543174552926e-09 -1.85986777702161e-09 -1.7901190036642e-09;-1.85986777702161e-09 7.82540023894543e-09 -1.8957321828871e-09;-1.7901190036642e-09 -1.8957321828871e-09 7.91264394645417e-09]  x1=[157.003522435008 1870.42653910552 1873.45371016496;314.159265358979 314.159265358979 314.159265358979;0.993627239752327 -0.794601201094145 -2.36380739557115]  x2=[157.003591771387 1870.42705832321 1873.45423118083;314.159265358979 314.159265358979 314.159265358979;0.993627050481464 -0.794601554289817 -2.36380775171645]  x3=[0.137255387038702 4.75851172908053 4.80280889948096;314.159265358979 314.159265358979 314.159265358979;0.992369761746573 -0.795597707622521 -2.36480477578221]  x4=[0.137254739530375 4.75851184516489 4.80280883918688;314.159265358979 314.159265358979 314.159265358979;0.994462989164056 -0.793939957467913 -2.36314560025828]  x5=1.3417561037125e-06  V1=ones(3,3)  V2=ones(3,3)  I1=ones(3,3)  I2=ones(3,3)  nHarmo=1  Measurements=None  Decoupling=off  VsMag0=0  VrMag0=0  VsAngle0=0  VrAngle0=0  IsMag0=0  IrMag0=0  IsAngle0=0  IrAngle0=0
      settings: SourceProductBaseCode=PS
  Line 48 : spsDistributedParametersLineLib/Distributed Parameters Line  Phases=3  Length=0.3  Frequency=50  Resistance=[0.80718830189013 0.0486237908083191 0.0486712220507153;0.0486237908083191 0.807093436079969 0.0486237934466192;0.0486712220507153 0.0486237934466192 0.80718830189013]  Inductance=[0.00279786707424938 0.00133270803418135 0.00132951476746136;0.00133270803418135 0.00279817608385787 0.00133799988507366;0.00132951476746136 0.00133799988507366 0.00279786707424938]  Capacitance=[7.73340098830622e-09 -1.79942827973291e-09 -1.73218055098733e-09;-1.79942827973291e-09 7.66505189233746e-09 -1.83375898618858e-09;-1.73218055098733e-09 -1.83375898618858e-09 7.749673531177e-09]  x1=[145.468327536726 1870.40466979634 1873.84374807451;314.159265358979 314.159265358979 314.159265358979;1.05282340055429 -0.798852585888835 -2.36802347632596]  x2=[145.468342149325 1870.40478533662 1873.84386402286;314.159265358979 314.159265358979 314.159265358979;1.05282334763226 -0.798852687387431 -2.36802357866973]  x3=[0.126748186136066 4.74586358195713 4.7908156688179;314.159265358979 314.159265358979 314.159265358979;1.05237514924046 -0.799204127438348 -2.36837531514946]  x4=[0.126748186850792 4.74586358220615 4.79081566884878;314.159265358979 314.159265358979 314.159265358979;1.05282334746568 -0.798852687304644 -2.36802357870356]  x5=1.42674452918375e-06  V1=ones(3,3)  V2=ones(3,3)  I1=ones(3,3)  I2=ones(3,3)  nHarmo=1  Measurements=None  Decoupling=off  VsMag0=0  VrMag0=0  VsAngle0=0  VrAngle0=0  IsMag0=0  IrMag0=0  IsAngle0=0  IrAngle0=0
      settings: SourceProductBaseCode=PS
  Line 49 : spsDistributedParametersLineLib/Distributed Parameters Line  Phases=3  Length=0.26  Frequency=50  Resistance=[0.646656091154803 0.0486237908083191 0.0486712220507153;0.0486237908083191 0.646561225344642 0.0486237934466192;0.0486712220507153 0.0486237934466192 0.646656091154803]  Inductance=[0.00282448912315926 0.00133270803418135 0.00132951476746136;0.00133270803418135 0.00282479813276775 0.00133799988507366;0.00132951476746136 0.00133799988507366 0.00282448912315926]  Capacitance=[7.89543174552926e-09 -1.85986777702161e-09 -1.7901190036642e-09;-1.85986777702161e-09 7.82540023894543e-09 -1.8957321828871e-09;-1.7901190036642e-09 -1.8957321828871e-09 7.91264394645417e-09]  x1=[157.003591771387 1870.42705832321 1873.45423118083;314.159265358979 314.159265358979 314.159265358979;0.993657201350978 -0.794577601404237 -2.36378377602942]  x2=[157.003603795903 1870.42714873223 1873.45432190852;314.159265358979 314.159265358979 314.159265358979;0.993657168322714 -0.79457766290275 -2.36378383804814]  x3=[0.137256364410891 4.75861973726091 4.80291864668589;314.159265358979 314.159265358979 314.159265358979;0.993265809141258 -0.794888553505063 -2.36409502407838]  x4=[0.137256364327264 4.7586197375134 4.80291864669776;314.159265358979 314.159265358979 314.159265358979;0.993657169784635 -0.794577662682177 -2.36378383811428]  x5=1.2457829052789e-06  V1=ones(3,3)  V2=ones(3,3)  I1=ones(3,3)  I2=ones(3,3)  nHarmo=1  Measurements=None  Decoupling=off  VsMag0=0  VrMag0=0  VsAngle0=0  VrAngle0=0  IsMag0=0  IrMag0=0  IsAngle0=0  IrAngle0=0
      settings: SourceProductBaseCode=PS
  Line 5 : spsDistributedParametersLineLib/Distributed Parameters Line  Phases=3  Length=1.62  Frequency=50  Resistance=[0.80718830189013 0.0486237908083191 0.0486712220507153;0.0486237908083191 0.807093436079969 0.0486237934466192;0.0486712220507153 0.0486237934466192 0.80718830189013]  Inductance=[0.00279786707424938 0.00133270803418135 0.00132951476746136;0.00133270803418135 0.00279817608385787 0.00133799988507366;0.00132951476746136 0.00133799988507366 0.00279786707424938]  Capacitance=[7.73340098830622e-09 -1.79942827973291e-09 -1.73218055098733e-09;-1.79942827973291e-09 7.66505189233746e-09 -1.83375898618858e-09;-1.73218055098733e-09 -1.83375898618858e-09 7.749673531177e-09]  x1=[145.403881243379 1871.83065606264 1875.27054919524;314.159265358979 314.159265358979 314.159265358979;1.05097169658375 -0.799784050170668 -2.36895977480215]  x2=[145.404373626476 1871.82870222726 1875.26860971114;314.159265358979 314.159265358979 314.159265358979;1.05097000693744 -0.799786871312773 -2.36896261343943]  x3=[0.12659763041855 4.73738017388756 4.78220271182601;314.159265358979 314.159265358979 314.159265358979;1.04837775462602 -0.80124661032781 -2.37042755738132]  x4=[0.126589908592683 4.74349977643528 4.78833319037071;314.159265358979 314.159265358979 314.159265358979;1.05114284656748 -0.800224500615607 -2.36939663689567]  x5=7.70442045759223e-06  V1=ones(3,3)  V2=ones(3,3)  I1=ones(3,3)  I2=ones(3,3)  nHarmo=1  Measurements=None  Decoupling=off  VsMag0=0  VrMag0=0  VsAngle0=0  VrAngle0=0  IsMag0=0  IrMag0=0  IsAngle0=0  IrAngle0=0
      settings: SourceProductBaseCode=PS
  Line 50 : spsDistributedParametersLineLib/Distributed Parameters Line  Phases=3  Length=0.02  Frequency=50  Resistance=[0.476003738225748 0.351747138225748 0.351747138225748;0.351747138225748 0.476003738225748 0.351747138225748;0.351747138225748 0.351747138225748 0.476003738225748]  Inductance=[0.000705954362986426 0.000459934243504405 0.000459934243504405;0.000459934243504405 0.000705954362986426 0.000459934243504405;0.000459934243504405 0.000459934243504405 0.000705954362986426]  Capacitance=[5.7561313269996e-07 -1.37543883484145e-07 -1.37543912800485e-07;-1.37543883484145e-07 5.75613027339387e-07 -1.37543875208088e-07;-1.37543912800485e-07 -1.37543875208088e-07 5.75613005057695e-07]  x1=[137.574444692689 1870.43882212508 1873.77325734619;314.159265358979 314.159265358979 314.159265358979;1.09270809996413 -0.712692745656771 -2.28193753109403]  x2=[137.574489867811 1870.43821958496 1873.77265383368;314.159265358979 314.159265358979 314.159265358979;1.09270730968355 -0.712693066295356 -2.2819378518865]  x3=[1.86991890132153 100.411822681867 100.590796811512;314.159265358979 314.159265358979 314.159265358979;1.09019006521673 -0.713384409075887 -2.28263020887654]  x4=[1.87005492031935 100.977854771022 101.157882985688;314.159265358979 314.159265358979 314.159265358979;1.09508626973486 -0.712088274375974 -2.28133205157039]  x5=4.42086352438419e-07  V1=ones(3,3)  V2=ones(3,3)  I1=ones(3,3)  I2=ones(3,3)  nHarmo=1  Measurements=None  Decoupling=off  VsMag0=0  VrMag0=0  VsAngle0=0  VrAngle0=0  IsMag0=0  IrMag0=0  IsAngle0=0  IrAngle0=0
      settings: SourceProductBaseCode=PS
  Line 51 : spsDistributedParametersLineLib/Distributed Parameters Line  Phases=3  Length=1.71  Frequency=50  Resistance=[0.646656091154803 0.0486237908083191 0.0486712220507153;0.0486237908083191 0.646561225344642 0.0486237934466192;0.0486712220507153 0.0486237934466192 0.646656091154803]  Inductance=[0.00282448912315926 0.00133270803418135 0.00132951476746136;0.00133270803418135 0.00282479813276775 0.00133799988507366;0.00132951476746136 0.00133799988507366 0.00282448912315926]  Capacitance=[7.89543174552926e-09 -1.85986777702161e-09 -1.7901190036642e-09;-1.85986777702161e-09 7.82540023894543e-09 -1.8957321828871e-09;-1.7901190036642e-09 -1.8957321828871e-09 7.91264394645417e-09]  x1=[156.985928700105 1870.65561643571 1873.68333104093;314.159265358979 314.159265358979 314.159265358979;0.991502773689873 -0.796147506064735 -2.36535605477794]  x2=[157.003138521445 1870.42576824092 1873.45293687261;314.159265358979 314.159265358979 314.159265358979;0.991479646513848 -0.796309731493859 -2.36551755186119]  x3=[0.138340565106398 4.46921400218089 4.51295496410893;314.159265358979 314.159265358979 314.159265358979;0.951365676191818 -0.81382209164731 -2.38293802132935]  x4=[0.136173136770703 5.03403297768704 5.07862893493702;314.159265358979 314.159265358979 314.159265358979;1.02966048429004 -0.78254070902644 -2.35181918227097]  x5=8.19341833856506e-06  V1=ones(3,3)  V2=ones(3,3)  I1=ones(3,3)  I2=ones(3,3)  nHarmo=1  Measurements=None  Decoupling=off  VsMag0=0  VrMag0=0  VsAngle0=0  VrAngle0=0  IsMag0=0  IrMag0=0  IsAngle0=0  IrAngle0=0
      settings: SourceProductBaseCode=PS
  Line 52 : spsDistributedParametersLineLib/Distributed Parameters Line  Phases=3  Length=0.02  Frequency=50  Resistance=[0.646656091154803 0.0486237908083191 0.0486712220507153;0.0486237908083191 0.646561225344642 0.0486237934466192;0.0486712220507153 0.0486237934466192 0.646656091154803]  Inductance=[0.00282448912315926 0.00133270803418135 0.00132951476746136;0.00133270803418135 0.00282479813276775 0.00133799988507366;0.00132951476746136 0.00133799988507366 0.00282448912315926]  Capacitance=[7.89543174552926e-09 -1.85986777702161e-09 -1.7901190036642e-09;-1.85986777702161e-09 7.82540023894543e-09 -1.8957321828871e-09;-1.7901190036642e-09 -1.8957321828871e-09 7.91264394645417e-09]  x1=[156.985928700105 1870.65561643571 1873.68333104093;314.159265358979 314.159265358979 314.159265358979;0.994046706264948 -0.794126518714268 -2.36333314359063]  x2=[156.985959812165 1870.65172693859 1873.67944036439;314.159265358979 314.159265358979 314.159265358979;0.994046720861649 -0.794127519134686 -2.3633341355245]  x3=[0.137643605644576 4.48381579328751 4.52766881331053;314.159265358979 314.159265358979 314.159265358979;0.988672414411024 -0.780469718118927 -2.34980880655497]  x4=[0.136874285038821 5.03797509708346 5.08276818204228;314.159265358979 314.159265358979 314.159265358979;0.999421029544864 -0.806304588337891 -2.37540395490189]  x5=9.5829454252223e-08  V1=ones(3,3)  V2=ones(3,3)  I1=ones(3,3)  I2=ones(3,3)  nHarmo=1  Measurements=None  Decoupling=off  VsMag0=0  VrMag0=0  VsAngle0=0  VrAngle0=0  IsMag0=0  IrMag0=0  IsAngle0=0  IrAngle0=0
      settings: SourceProductBaseCode=PS
  Line 53 : spsDistributedParametersLineLib/Distributed Parameters Line  Phases=3  Length=0.02  Frequency=50  Resistance=[0.646656091154803 0.0486237908083191 0.0486712220507153;0.0486237908083191 0.646561225344642 0.0486237934466192;0.0486712220507153 0.0486237934466192 0.646656091154803]  Inductance=[0.00282448912315926 0.00133270803418135 0.00132951476746136;0.00133270803418135 0.00282479813276775 0.00133799988507366;0.00132951476746136 0.00133799988507366 0.00282448912315926]  Capacitance=[7.89543174552926e-09 -1.85986777702161e-09 -1.7901190036642e-09;-1.85986777702161e-09 7.82540023894543e-09 -1.8957321828871e-09;-1.7901190036642e-09 -1.8957321828871e-09 7.91264394645417e-09]  x1=[156.985690078776 1870.66214770345 1873.68986970646;314.159265358979 314.159265358979 314.159265358979;0.994046979293558 -0.794123589324975 -2.36333023093607]  x2=[156.985928700105 1870.65561643571 1873.68333104093;314.159265358979 314.159265358979 314.159265358979;0.994046706264948 -0.794126518714268 -2.36333314359063]  x3=[0.138869971325529 4.20027097663954 4.2436955310976;314.159265358979 314.159265358979 314.159265358979;0.948679539268259 -0.798401551961891 -2.36764886843252]  x4=[0.135932390680231 5.32082307479713 5.36605428701396;314.159265358979 314.159265358979 314.159265358979;1.04036482435181 -0.790770578482962 -2.35993892382111]  x5=9.5829454252223e-08  V1=ones(3,3)  V2=ones(3,3)  I1=ones(3,3)  I2=ones(3,3)  nHarmo=1  Measurements=None  Decoupling=off  VsMag0=0  VrMag0=0  VsAngle0=0  VrAngle0=0  IsMag0=0  IrMag0=0  IsAngle0=0  IrAngle0=0
      settings: SourceProductBaseCode=PS
  Line 54 : spsDistributedParametersLineLib/Distributed Parameters Line  Phases=3  Length=1.1501  Frequency=50  Resistance=[0.646656091154803 0.0486237908083191 0.0486712220507153;0.0486237908083191 0.646561225344642 0.0486237934466192;0.0486712220507153 0.0486237934466192 0.646656091154803]  Inductance=[0.00282448912315926 0.00133270803418135 0.00132951476746136;0.00133270803418135 0.00282479813276775 0.00133799988507366;0.00132951476746136 0.00133799988507366 0.00282448912315926]  Capacitance=[7.89543174552926e-09 -1.85986777702161e-09 -1.7901190036642e-09;-1.85986777702161e-09 7.82540023894543e-09 -1.8957321828871e-09;-1.7901190036642e-09 -1.8957321828871e-09 7.91264394645417e-09]  x1=[156.985690078776 1870.66214770345 1873.68986970646;314.159265358979 314.159265358979 314.159265358979;0.992345856096462 -0.795475019978681 -2.36468294805606]  x2=[156.988471913493 1870.41245037229 1873.44022082325;314.159265358979 314.159265358979 314.159265358979;0.992342946223815 -0.795525304703451 -2.36473276305115]  x3=[0.137504455607943 4.46458724842743 4.5082954589291;314.159265358979 314.159265358979 314.159265358979;0.982260156599664 -0.775644743771865 -2.34506498496499]  x4=[0.136872278775326 5.04532904941927 5.09004421701944;314.159265358979 314.159265358979 314.159265358979;1.00073967253617 -0.814366605601552 -2.38340400146666]  x5=5.51067276677408e-06  V1=ones(3,3)  V2=ones(3,3)  I1=ones(3,3)  I2=ones(3,3)  nHarmo=1  Measurements=None  Decoupling=off  VsMag0=0  VrMag0=0  VsAngle0=0  VrAngle0=0  IsMag0=0  IrMag0=0  IsAngle0=0  IrAngle0=0
      settings: SourceProductBaseCode=PS
  Line 55 : spsDistributedParametersLineLib/Distributed Parameters Line  Phases=3  Length=0.18999  Frequency=50  Resistance=[0.646656091154803 0.0486237908083191 0.0486712220507153;0.0486237908083191 0.646561225344642 0.0486237934466192;0.0486712220507153 0.0486237934466192 0.646656091154803]  Inductance=[0.00282448912315926 0.00133270803418135 0.00132951476746136;0.00133270803418135 0.00282479813276775 0.00133799988507366;0.00132951476746136 0.00133799988507366 0.00282448912315926]  Capacitance=[7.89543174552926e-09 -1.85986777702161e-09 -1.7901190036642e-09;-1.85986777702161e-09 7.82540023894543e-09 -1.8957321828871e-09;-1.7901190036642e-09 -1.8957321828871e-09 7.91264394645417e-09]  x1=[156.988471913493 1870.41245037229 1873.44022082325;314.159265358979 314.159265358979 314.159265358979;0.993788185930712 -0.79437715667679 -2.36358352206887]  x2=[156.988593047209 1870.39798158952 1873.425749003;314.159265358979 314.159265358979 314.159265358979;0.993788205136645 -0.794380693022773 -2.36358702761596]  x3=[0.13739063258583 4.6520170072329 4.6961406173977;314.159265358979 314.159265358979 314.159265358979;0.991397075455949 -0.788928575293768 -2.35818753508934]  x4=[0.137105798694173 4.86601210818658 4.91050003883281;314.159265358979 314.159265358979 314.159265358979;0.995897988015014 -0.79981179908118 -2.36896985165834]  x5=9.10331900668992e-07  V1=ones(3,3)  V2=ones(3,3)  I1=ones(3,3)  I2=ones(3,3)  nHarmo=1  Measurements=None  Decoupling=off  VsMag0=0  VrMag0=0  VsAngle0=0  VrAngle0=0  IsMag0=0  IrMag0=0  IsAngle0=0  IrAngle0=0
      settings: SourceProductBaseCode=PS
  Line 56 : spsDistributedParametersLineLib/Distributed Parameters Line  Phases=3  Length=0.34002  Frequency=50  Resistance=[0.646656091154803 0.0486237908083191 0.0486712220507153;0.0486237908083191 0.646561225344642 0.0486237934466192;0.0486712220507153 0.0486237934466192 0.646656091154803]  Inductance=[0.00282448912315926 0.00133270803418135 0.00132951476746136;0.00133270803418135 0.00282479813276775 0.00133799988507366;0.00132951476746136 0.00133799988507366 0.00282448912315926]  Capacitance=[7.89543174552926e-09 -1.85986777702161e-09 -1.7901190036642e-09;-1.85986777702161e-09 7.82540023894543e-09 -1.8957321828871e-09;-1.7901190036642e-09 -1.8957321828871e-09 7.91264394645417e-09]  x1=[156.988471913493 1870.41245037229 1873.44022082325;314.159265358979 314.159265358979 314.159265358979;0.993562347940038 -0.794556570127791 -2.36376310630877]  x2=[156.988975951439 1870.3637600093 1873.391547512;314.159265358979 314.159265358979 314.159265358979;0.993561732405747 -0.794564590116352 -2.3637710381212]  x3=[0.137414126863348 4.57482139776403 4.61878458565134;314.159265358979 314.159265358979 314.159265358979;0.987587170478807 -0.779305184941553 -2.34866036547067]  x4=[0.137066400826516 4.94240323337853 4.98701486588173;314.159265358979 314.159265358979 314.159265358979;0.999039563065006 -0.809072845773536 -2.37815027908177]  x5=1.62919655174204e-06  V1=ones(3,3)  V2=ones(3,3)  I1=ones(3,3)  I2=ones(3,3)  nHarmo=1  Measurements=None  Decoupling=off  VsMag0=0  VrMag0=0  VsAngle0=0  VrAngle0=0  IsMag0=0  IrMag0=0  IsAngle0=0  IrAngle0=0
      settings: SourceProductBaseCode=PS
  Line 57 : spsDistributedParametersLineLib/Distributed Parameters Line  Phases=3  Length=0.12001  Frequency=50  Resistance=[0.646656091154803 0.0486237908083191 0.0486712220507153;0.0486237908083191 0.646561225344642 0.0486237934466192;0.0486712220507153 0.0486237934466192 0.646656091154803]  Inductance=[0.00282448912315926 0.00133270803418135 0.00132951476746136;0.00133270803418135 0.00282479813276775 0.00133799988507366;0.00132951476746136 0.00133799988507366 0.00282448912315926]  Capacitance=[7.89543174552926e-09 -1.85986777702161e-09 -1.7901190036642e-09;-1.85986777702161e-09 7.82540023894543e-09 -1.8957321828871e-09;-1.7901190036642e-09 -1.8957321828871e-09 7.91264394645417e-09]  x1=[156.988975951439 1870.3637600093 1873.391547512;314.159265358979 314.159265358979 314.159265358979;0.993892910279026 -0.794301491047135 -2.3635076886003]  x2=[156.989018723904 1870.35841182278 1873.38620055605;314.159265358979 314.159265358979 314.159265358979;0.993892881078001 -0.794302352158879 -2.36350853952306]  x3=[0.13730963510434 4.70229325275725 4.74650474904483;314.159265358979 314.159265358979 314.159265358979;0.992472672388493 -0.789623905868706 -2.3588717120682]  x4=[0.137196507570563 4.81623529869186 4.86064701141231;314.159265358979 314.159265358979 314.159265358979;0.995133562721261 -0.799011087333926 -2.36817760942924]  x5=5.75024640240464e-07  V1=ones(3,3)  V2=ones(3,3)  I1=ones(3,3)  I2=ones(3,3)  nHarmo=1  Measurements=None  Decoupling=off  VsMag0=0  VrMag0=0  VsAngle0=0  VrAngle0=0  IsMag0=0  IrMag0=0  IsAngle0=0  IrAngle0=0
      settings: SourceProductBaseCode=PS
  Line 58 : spsDistributedParametersLineLib/Distributed Parameters Line  Phases=3  Length=0.82  Frequency=50  Resistance=[0.646656091154803 0.0486237908083191 0.0486712220507153;0.0486237908083191 0.646561225344642 0.0486237934466192;0.0486712220507153 0.0486237934466192 0.646656091154803]  Inductance=[0.00282448912315926 0.00133270803418135 0.00132951476746136;0.00133270803418135 0.00282479813276775 0.00133799988507366;0.00132951476746136 0.00133799988507366 0.00282448912315926]  Capacitance=[7.89543174552926e-09 -1.85986777702161e-09 -1.7901190036642e-09;-1.85986777702161e-09 7.82540023894543e-09 -1.8957321828871e-09;-1.7901190036642e-09 -1.8957321828871e-09 7.91264394645417e-09]  x1=[156.988975951439 1870.3637600093 1873.391547512;314.159265358979 314.159265358979 314.159265358979;0.992839225448715 -0.795138574440895 -2.36434556883818]  x2=[156.989712560161 1870.28147669467 1873.30929195291;314.159265358979 314.159265358979 314.159265358979;0.99283845337962 -0.795151078045809 -2.36435792132225]  x3=[0.137324593722968 4.62884016433479 4.67286170028926;314.159265358979 314.159265358979 314.159265358979;0.988792327997037 -0.784402769473725 -2.35371209019738]  x4=[0.137090046122937 4.8823583417935 4.92682631386947;314.159265358979 314.159265358979 314.159265358979;0.995656719570803 -0.806284511402061 -2.37539946600967]  x5=3.92900762434114e-06  V1=ones(3,3)  V2=ones(3,3)  I1=ones(3,3)  I2=ones(3,3)  nHarmo=1  Measurements=None  Decoupling=off  VsMag0=0  VrMag0=0  VsAngle0=0  VrAngle0=0  IsMag0=0  IrMag0=0  IsAngle0=0  IrAngle0=0
      settings: SourceProductBaseCode=PS
  Line 59 : spsDistributedParametersLineLib/Distributed Parameters Line  Phases=3  Length=1.11  Frequency=50  Resistance=[0.646656091154803 0.0486237908083191 0.0486712220507153;0.0486237908083191 0.646561225344642 0.0486237934466192;0.0486712220507153 0.0486237934466192 0.646656091154803]  Inductance=[0.00282448912315926 0.00133270803418135 0.00132951476746136;0.00133270803418135 0.00282479813276775 0.00133799988507366;0.00132951476746136 0.00133799988507366 0.00282448912315926]  Capacitance=[7.89543174552926e-09 -1.85986777702161e-09 -1.7901190036642e-09;-1.85986777702161e-09 7.82540023894543e-09 -1.8957321828871e-09;-1.7901190036642e-09 -1.8957321828871e-09 7.91264394645417e-09]  x1=[156.969311652266 1871.26228409423 1874.29035744908;314.159265358979 314.159265358979 314.159265358979;0.992425418156558 -0.795213726785954 -2.36442297128229]  x2=[156.985690078776 1870.66214770345 1873.68986970646;314.159265358979 314.159265358979 314.159265358979;0.992406218046912 -0.795427066373501 -2.36463494880245]  x3=[0.139180567812168 3.90616528319199 3.94898640445935;314.159265358979 314.159265358979 314.159265358979;0.935548537651522 -0.778715012494147 -2.34823333916885]  x4=[0.135615661528512 5.60555847786131 5.65118056636526;314.159265358979 314.159265358979 314.159265358979;1.04908643030897 -0.808017981608835 -2.37704488638862]  x5=5.31853471099837e-06  V1=ones(3,3)  V2=ones(3,3)  I1=ones(3,3)  I2=ones(3,3)  nHarmo=1  Measurements=None  Decoupling=off  VsMag0=0  VrMag0=0  VsAngle0=0  VrAngle0=0  IsMag0=0  IrMag0=0  IsAngle0=0  IrAngle0=0
      settings: SourceProductBaseCode=PS
  Line 6 : spsDistributedParametersLineLib/Distributed Parameters Line  Phases=3  Length=0.54002  Frequency=50  Resistance=[0.646656091154803 0.0486237908083191 0.0486712220507153;0.0486237908083191 0.646561225344642 0.0486237934466192;0.0486712220507153 0.0486237934466192 0.646656091154803]  Inductance=[0.00282448912315926 0.00133270803418135 0.00132951476746136;0.00133270803418135 0.00282479813276775 0.00133799988507366;0.00132951476746136 0.00133799988507366 0.00282448912315926]  Capacitance=[7.89543174552926e-09 -1.85986777702161e-09 -1.7901190036642e-09;-1.85986777702161e-09 7.82540023894543e-09 -1.8957321828871e-09;-1.7901190036642e-09 -1.8957321828871e-09 7.91264394645417e-09]  x1=[156.941937925151 1872.28617161936 1875.3144168448;314.159265358979 314.159265358979 314.159265358979;0.993352806573319 -0.794142116591057 -2.36335299433864]  x2=[156.952553131653 1871.85294613081 1874.88113522112;314.159265358979 314.159265358979 314.159265358979;0.993327173464728 -0.794297274827073 -2.36350720752784]  x3=[0.13814585803759 3.49707531833845 3.53952538969516;314.159265358979 314.159265358979 314.159265358979;0.911794162840298 -0.767167938690226 -2.33703934239198]  x4=[0.13714327670001 6.0275488187452 6.07364321014341;314.159265358979 314.159265358979 314.159265358979;1.07466734685282 -0.810423640238523 -2.3793202104826]  x5=2.58749109426427e-06  V1=ones(3,3)  V2=ones(3,3)  I1=ones(3,3)  I2=ones(3,3)  nHarmo=1  Measurements=None  Decoupling=off  VsMag0=0  VrMag0=0  VsAngle0=0  VrAngle0=0  IsMag0=0  IrMag0=0  IsAngle0=0  IrAngle0=0
      settings: SourceProductBaseCode=PS
  Line 60 : spsDistributedParametersLineLib/Distributed Parameters Line  Phases=3  Length=0.20999  Frequency=50  Resistance=[0.646656091154803 0.0486237908083191 0.0486712220507153;0.0486237908083191 0.646561225344642 0.0486237934466192;0.0486712220507153 0.0486237934466192 0.646656091154803]  Inductance=[0.00282448912315926 0.00133270803418135 0.00132951476746136;0.00133270803418135 0.00282479813276775 0.00133799988507366;0.00132951476746136 0.00133799988507366 0.00282448912315926]  Capacitance=[7.89543174552926e-09 -1.85986777702161e-09 -1.7901190036642e-09;-1.85986777702161e-09 7.82540023894543e-09 -1.8957321828871e-09;-1.7901190036642e-09 -1.8957321828871e-09 7.91264394645417e-09]  x1=[156.969311652266 1871.26228409423 1874.29035744908;314.159265358979 314.159265358979 314.159265358979;0.993780190202057 -0.794137449374537 -2.36334566933099]  x2=[156.970409117165 1871.27185672426 1874.29988279924;314.159265358979 314.159265358979 314.159265358979;0.993778570434781 -0.794143963536377 -2.36335217813013]  x3=[0.137769737240705 4.76197690124946 4.8063290698763;314.159265358979 314.159265358979 314.159265358979;0.97318753554145 -0.814644076950066 -2.38368991304786]  x4=[0.136748415959453 4.7620571138886 4.80633597633718;314.159265358979 314.159265358979 314.159265358979;1.01420775301836 -0.773888815975203 -2.34325933940151]  x5=1.00616135492121e-06  V1=ones(3,3)  V2=ones(3,3)  I1=ones(3,3)  I2=ones(3,3)  nHarmo=1  Measurements=None  Decoupling=off  VsMag0=0  VrMag0=0  VsAngle0=0  VrAngle0=0  IsMag0=0  IrMag0=0  IsAngle0=0  IrAngle0=0
      settings: SourceProductBaseCode=PS
  Line 61 : spsDistributedParametersLineLib/Distributed Parameters Line  Phases=3  Length=0.23002  Frequency=50  Resistance=[0.476003738225748 0.351747138225748 0.351747138225748;0.351747138225748 0.476003738225748 0.351747138225748;0.351747138225748 0.351747138225748 0.476003738225748]  Inductance=[0.000705954362986426 0.000459934243504405 0.000459934243504405;0.000459934243504405 0.000705954362986426 0.000459934243504405;0.000459934243504405 0.000459934243504405 0.000705954362986426]  Capacitance=[5.7561313269996e-07 -1.37543883484145e-07 -1.37543912800485e-07;-1.37543883484145e-07 5.75613027339387e-07 -1.37543875208088e-07;-1.37543912800485e-07 -1.37543875208088e-07 5.75613005057695e-07]  x1=[137.528209197329 1871.28510469667 1874.62023885939;314.159265358979 314.159265358979 314.159265358979;1.09132009689668 -0.713194654433905 -2.28244149466725]  x2=[137.528384644336 1871.28596192538 1874.62109761565;314.159265358979 314.159265358979 314.159265358979;1.09131715091783 -0.713195390905214 -2.28244223113844]  x3=[1.86463978743112 100.634344717252 100.813694441808;314.159265358979 314.159265358979 314.159265358979;1.08972130165068 -0.714152202128325 -2.28339904226416]  x4=[1.86463979041211 100.634344730539 100.813694461429;314.159265358979 314.159265358979 314.159265358979;1.09131715076261 -0.713195390881674 -2.28244223113823]  x5=5.08443513939426e-06  V1=ones(3,3)  V2=ones(3,3)  I1=ones(3,3)  I2=ones(3,3)  nHarmo=1  Measurements=None  Decoupling=off  VsMag0=0  VrMag0=0  VsAngle0=0  VrAngle0=0  IsMag0=0  IrMag0=0  IsAngle0=0  IrAngle0=0
      settings: SourceProductBaseCode=PS
  Line 62 : spsDistributedParametersLineLib/Distributed Parameters Line  Phases=3  Length=0.24002  Frequency=50  Resistance=[0.646656091154803 0.0486237908083191 0.0486712220507153;0.0486237908083191 0.646561225344642 0.0486237934466192;0.0486712220507153 0.0486237934466192 0.646656091154803]  Inductance=[0.00282448912315926 0.00133270803418135 0.00132951476746136;0.00133270803418135 0.00282479813276775 0.00133799988507366;0.00132951476746136 0.00133799988507366 0.00282448912315926]  Capacitance=[7.89543174552926e-09 -1.85986777702161e-09 -1.7901190036642e-09;-1.85986777702161e-09 7.82540023894543e-09 -1.8957321828871e-09;-1.7901190036642e-09 -1.8957321828871e-09 7.91264394645417e-09]  x1=[128.511435472042 6087.2507644917 6088.48631290335;314.159265358979 314.159265358979 314.159265358979;0.929408777987223 -0.367330784299461 -1.9386649817606]  x2=[130.220285493139 5778.64498281735 5780.03432490305;314.159265358979 314.159265358979 314.159265358979;0.934349717757181 -0.376767392613757 -1.94806911957124]  x3=[4.13276160379404 1704.45563982871 1707.89099224653;314.159265358979 314.159265358979 314.159265358979;0.145731073176809 2.27859764983878 0.709964360097096]  x4=[3.97613598042252 1731.13755761104 1734.82190518313;314.159265358979 314.159265358979 314.159265358979;-3.03612130128317 -0.854773574360713 -2.42340106682433]  x5=1.15004928048093e-06  V1=ones(3,3)  V2=ones(3,3)  I1=ones(3,3)  I2=ones(3,3)  nHarmo=1  Measurements=None  Decoupling=off  VsMag0=0  VrMag0=0  VsAngle0=0  VrAngle0=0  IsMag0=0  IrMag0=0  IsAngle0=0  IrAngle0=0
      settings: SourceProductBaseCode=PS
  Line 63 : spsDistributedParametersLineLib/Distributed Parameters Line  Phases=3  Length=0.02  Frequency=50  Resistance=[0.646656091154803 0.0486237908083191 0.0486712220507153;0.0486237908083191 0.646561225344642 0.0486237934466192;0.0486712220507153 0.0486237934466192 0.646656091154803]  Inductance=[0.00282448912315926 0.00133270803418135 0.00132951476746136;0.00133270803418135 0.00282479813276775 0.00133799988507366;0.00132951476746136 0.00133799988507366 0.00282448912315926]  Capacitance=[7.89543174552926e-09 -1.85986777702161e-09 -1.7901190036642e-09;-1.85986777702161e-09 7.82540023894543e-09 -1.8957321828871e-09;-1.7901190036642e-09 -1.8957321828871e-09 7.91264394645417e-09]  x1=[128.511435472042 6087.2507644917 6088.48631290335;314.159265358979 314.159265358979 314.159265358979;0.929739970913358 -0.367067673271739 -1.93840162026981]  x2=[128.511465050914 6087.24653377354 6088.48208904981;314.159265358979 314.159265358979 314.159265358979;0.929740052043623 -0.367067832371503 -1.93840177699211]  x3=[0.112930304629798 15.2334588743258 15.3554641802182;314.159265358979 314.159265358979 314.159265358979;0.924286059985457 -0.359082066111968 -1.93048166948198]  x4=[0.111794972828191 15.7495515869088 15.8718295711754;314.159265358979 314.159265358979 314.159265358979;0.935219092517071 -0.374815278772237 -1.94608760728751]  x5=9.5829454252223e-08  V1=ones(3,3)  V2=ones(3,3)  I1=ones(3,3)  I2=ones(3,3)  nHarmo=1  Measurements=None  Decoupling=off  VsMag0=0  VrMag0=0  VsAngle0=0  VrAngle0=0  IsMag0=0  IrMag0=0  IsAngle0=0  IrAngle0=0
      settings: SourceProductBaseCode=PS
  Line 64 : spsDistributedParametersLineLib/Distributed Parameters Line  Phases=3  Length=0.5  Frequency=50  Resistance=[0.646656091154803 0.0486237908083191 0.0486712220507153;0.0486237908083191 0.646561225344642 0.0486237934466192;0.0486712220507153 0.0486237934466192 0.646656091154803]  Inductance=[0.00282448912315926 0.00133270803418135 0.00132951476746136;0.00133270803418135 0.00282479813276775 0.00133799988507366;0.00132951476746136 0.00133799988507366 0.00282448912315926]  Capacitance=[7.89543174552926e-09 -1.85986777702161e-09 -1.7901190036642e-09;-1.85986777702161e-09 7.82540023894543e-09 -1.8957321828871e-09;-1.7901190036642e-09 -1.8957321828871e-09 7.91264394645417e-09]  x1=[124.961335478387 6731.72489781448 6732.63007753465;314.159265358979 314.159265358979 314.159265358979;0.918289442556433 -0.350762434012303 -1.92215326653817]  x2=[128.511435472042 6087.2507644917 6088.48631290335;314.159265358979 314.159265358979 314.159265358979;0.929017433850615 -0.367641681513292 -1.93897617492657]  x3=[4.13193061749226 1703.09793771917 1706.51771590025;314.159265358979 314.159265358979 314.159265358979;0.14458384771086 2.27769507565844 0.709060482215971]  x4=[3.97727261257366 1731.70597731402 1735.39315342234;314.159265358979 314.159265358979 314.159265358979;-3.03614776673163 -0.854791680114883 -2.42341961773323]  x5=2.39573635630557e-06  V1=ones(3,3)  V2=ones(3,3)  I1=ones(3,3)  I2=ones(3,3)  nHarmo=1  Measurements=None  Decoupling=off  VsMag0=0  VrMag0=0  VsAngle0=0  VrAngle0=0  IsMag0=0  IrMag0=0  IsAngle0=0  IrAngle0=0
      settings: SourceProductBaseCode=PS
  Line 65 : spsDistributedParametersLineLib/Distributed Parameters Line  Phases=3  Length=0.23  Frequency=50  Resistance=[0.646656091154803 0.0486237908083191 0.0486712220507153;0.0486237908083191 0.646561225344642 0.0486237934466192;0.0486712220507153 0.0486237934466192 0.646656091154803]  Inductance=[0.00282448912315926 0.00133270803418135 0.00132951476746136;0.00133270803418135 0.00282479813276775 0.00133799988507366;0.00132951476746136 0.00133799988507366 0.00282448912315926]  Capacitance=[7.89543174552926e-09 -1.85986777702161e-09 -1.7901190036642e-09;-1.85986777702161e-09 7.82540023894543e-09 -1.8957321828871e-09;-1.7901190036642e-09 -1.8957321828871e-09 7.91264394645417e-09]  x1=[123.330928212769 7029.08323802527 7029.83225044454;314.159265358979 314.159265358979 314.159265358979;0.913546888273094 -0.343705486227043 -1.91511796926076]  x2=[124.961335478387 6731.72489781448 6732.63007753465;314.159265358979 314.159265358979 314.159265358979;0.918695869654224 -0.350439554376429 -1.92183007954375]  x3=[4.13753979984166 1704.84276222541 1708.26096416918;314.159265358979 314.159265358979 314.159265358979;0.144587811273089 2.2778008480669 0.709163301450696]  x4=[3.98478861564218 1735.3696271943 1739.07363692074;314.159265358979 314.159265358979 314.159265358979;-3.0349887618442 -0.853825919557586 -2.42245593003315]  x5=1.10203872390056e-06  V1=ones(3,3)  V2=ones(3,3)  I1=ones(3,3)  I2=ones(3,3)  nHarmo=1  Measurements=None  Decoupling=off  VsMag0=0  VrMag0=0  VsAngle0=0  VrAngle0=0  IsMag0=0  IrMag0=0  IsAngle0=0  IrAngle0=0
      settings: SourceProductBaseCode=PS
  Line 66 : spsDistributedParametersLineLib/Distributed Parameters Line  Phases=3  Length=1.62  Frequency=50  Resistance=[0.80718830189013 0.0486237908083191 0.0486712220507153;0.0486237908083191 0.807093436079969 0.0486237934466192;0.0486712220507153 0.0486237934466192 0.80718830189013]  Inductance=[0.00279786707424938 0.00133270803418135 0.00132951476746136;0.00133270803418135 0.00279817608385787 0.00133799988507366;0.00132951476746136 0.00133799988507366 0.00279786707424938]  Capacitance=[7.73340098830622e-09 -1.79942827973291e-09 -1.73218055098733e-09;-1.79942827973291e-09 7.66505189233746e-09 -1.83375898618858e-09;-1.73218055098733e-09 -1.83375898618858e-09 7.749673531177e-09]  x1=[68.8505273707824 7029.13559115613 7030.04641388033;314.159265358979 314.159265358979 314.159265358979;0.99116713492676 -0.349635816791053 -1.92101569242422]  x2=[68.8509420493051 7029.1304023138 7030.04126565758;314.159265358979 314.159265358979 314.159265358979;0.991167205564645 -0.349639383370093 -1.92101927574673]  x3=[0.0600067011375012 17.7892928615833 17.9269890882169;314.159265358979 314.159265358979 314.159265358979;0.9880234879469 -0.351316685218554 -1.92269995236461]  x4=[0.0598809827024679 17.8135057457614 17.9512103756787;314.159265358979 314.159265358979 314.159265358979;0.991893724377729 -0.349859035987474 -1.92123714901327]  x5=7.70442045759223e-06  V1=ones(3,3)  V2=ones(3,3)  I1=ones(3,3)  I2=ones(3,3)  nHarmo=1  Measurements=None  Decoupling=off  VsMag0=0  VrMag0=0  VsAngle0=0  VrAngle0=0  IsMag0=0  IrMag0=0  IsAngle0=0  IrAngle0=0
      settings: SourceProductBaseCode=PS
  Line 67 : spsDistributedParametersLineLib/Distributed Parameters Line  Phases=3  Length=0.54002  Frequency=50  Resistance=[0.646656091154803 0.0486237908083191 0.0486712220507153;0.0486237908083191 0.646561225344642 0.0486237934466192;0.0486712220507153 0.0486237934466192 0.646656091154803]  Inductance=[0.00282448912315926 0.00133270803418135 0.00132951476746136;0.00133270803418135 0.00282479813276775 0.00133799988507366;0.00132951476746136 0.00133799988507366 0.00282448912315926]  Capacitance=[7.89543174552926e-09 -1.85986777702161e-09 -1.7901190036642e-09;-1.85986777702161e-09 7.82540023894543e-09 -1.8957321828871e-09;-1.7901190036642e-09 -1.8957321828871e-09 7.91264394645417e-09]  x1=[119.515985029828 7728.34046847707 7728.71589031762;314.159265358979 314.159265358979 314.159265358979;0.900440647369374 -0.330301808625459 -1.90175836326545]  x2=[123.330928212769 7029.08323802527 7029.83225044454;314.159265358979 314.159265358979 314.159265358979;0.913080219647694 -0.344076223800056 -1.91548905974969]  x3=[4.13590944286567 1703.02533181456 1706.42614100255;314.159265358979 314.159265358979 314.159265358979;0.143271444471818 2.27679930216628 0.708160874656106]  x4=[3.98521688937633 1735.55637663456 1739.26212526831;314.159265358979 314.159265358979 314.159265358979;-3.03514705854021 -0.85390547195606 -2.42253547799819]  x5=2.58749109426427e-06  V1=ones(3,3)  V2=ones(3,3)  I1=ones(3,3)  I2=ones(3,3)  nHarmo=1  Measurements=None  Decoupling=off  VsMag0=0  VrMag0=0  VsAngle0=0  VrAngle0=0  IsMag0=0  IrMag0=0  IsAngle0=0  IrAngle0=0
      settings: SourceProductBaseCode=PS
  Line 68 : spsDistributedParametersLineLib/Distributed Parameters Line  Phases=3  Length=0.13998  Frequency=50  Resistance=[0.646656091154803 0.0486237908083191 0.0486712220507153;0.0486237908083191 0.646561225344642 0.0486237934466192;0.0486712220507153 0.0486237934466192 0.646656091154803]  Inductance=[0.00282448912315926 0.00133270803418135 0.00132951476746136;0.00133270803418135 0.00282479813276775 0.00133799988507366;0.00132951476746136 0.00133799988507366 0.00282448912315926]  Capacitance=[7.89543174552926e-09 -1.85986777702161e-09 -1.7901190036642e-09;-1.85986777702161e-09 7.82540023894543e-09 -1.8957321828871e-09;-1.7901190036642e-09 -1.8957321828871e-09 7.91264394645417e-09]  x1=[119.515985029828 7728.34046847707 7728.71589031762;314.159265358979 314.159265358979 314.159265358979;0.901042821799749 -0.329823420590145 -1.9012795198386]  x2=[119.517355908403 7728.14805305697 7728.52379087702;314.159265358979 314.159265358979 314.159265358979;0.901047863456709 -0.329830166315231 -1.90128617759525]  x3=[0.108736278887793 17.9558118491362 18.1070189349492;314.159265358979 314.159265358979 314.159265358979;0.865186488596922 -0.289142525414918 -1.86095767255852]  x4=[0.100389452744455 21.4004081783762 21.5529089952785;314.159265358979 314.159265358979 314.159265358979;0.939667617019688 -0.364113672479407 -1.93531226424949]  x5=6.70710350311308e-07  V1=ones(3,3)  V2=ones(3,3)  I1=ones(3,3)  I2=ones(3,3)  nHarmo=1  Measurements=None  Decoupling=off  VsMag0=0  VrMag0=0  VsAngle0=0  VrAngle0=0  IsMag0=0  IrMag0=0  IsAngle0=0  IrAngle0=0
      settings: SourceProductBaseCode=PS
  Line 69 : spsDistributedParametersLineLib/Distributed Parameters Line  Phases=3  Length=0.14997  Frequency=50  Resistance=[0.476003738225748 0.351747138225748 0.351747138225748;0.351747138225748 0.476003738225748 0.351747138225748;0.351747138225748 0.351747138225748 0.476003738225748]  Inductance=[0.000705954362986426 0.000459934243504405 0.000459934243504405;0.000459934243504405 0.000705954362986426 0.000459934243504405;0.000459934243504405 0.000459934243504405 0.000705954362986426]  Capacitance=[5.7561313269996e-07 -1.37543883484145e-07 -1.37543912800485e-07;-1.37543883484145e-07 5.75613027339387e-07 -1.37543875208088e-07;-1.37543912800485e-07 -1.37543875208088e-07 5.75613005057695e-07]  x1=[19.3111806124746 7729.26802052135 7729.66504691682;314.159265358979 314.159265358979 314.159265358979;1.08385382298343 -0.24863829431125 -1.81994565937989]  x2=[19.3111910867685 7729.22589198719 7729.62291621826;314.159265358979 314.159265358979 314.159265358979;1.08385257116578 -0.24863879846935 -1.81994616353795]  x3=[0.262077498535969 414.110557607853 414.13179693651;314.159265358979 314.159265358979 314.159265358979;1.08281191585243 -0.246868395657308 -1.81817576048844]  x4=[0.26207744147434 417.554804879825 417.576221144918;314.159265358979 314.159265358979 314.159265358979;1.08385241937237 -0.251015746191439 -1.82232311144601]  x5=3.31498451375949e-06  V1=ones(3,3)  V2=ones(3,3)  I1=ones(3,3)  I2=ones(3,3)  nHarmo=1  Measurements=None  Decoupling=off  VsMag0=0  VrMag0=0  VsAngle0=0  VrAngle0=0  IsMag0=0  IrMag0=0  IsAngle0=0  IrAngle0=0
      settings: SourceProductBaseCode=PS
  Line 7 : spsDistributedParametersLineLib/Distributed Parameters Line  Phases=3  Length=0.13998  Frequency=50  Resistance=[0.646656091154803 0.0486237908083191 0.0486712220507153;0.0486237908083191 0.646561225344642 0.0486237934466192;0.0486712220507153 0.0486237934466192 0.646656091154803]  Inductance=[0.00282448912315926 0.00133270803418135 0.00132951476746136;0.00133270803418135 0.00282479813276775 0.00133799988507366;0.00132951476746136 0.00133799988507366 0.00282448912315926]  Capacitance=[7.89543174552926e-09 -1.85986777702161e-09 -1.7901190036642e-09;-1.85986777702161e-09 7.82540023894543e-09 -1.8957321828871e-09;-1.7901190036642e-09 -1.8957321828871e-09 7.91264394645417e-09]  x1=[156.941937925151 1872.28617161936 1875.3144168448;314.159265358979 314.159265358979 314.159265358979;0.993954981003694 -0.793663728555743 -2.36287415091179]  x2=[158.223145454858 1725.00698317546 1727.90241824334;314.159265358979 314.159265358979 314.159265358979;0.995830979047761 -0.853534867999568 -2.42237155934626]  x3=[5.092359281985 1708.50440543022 1711.28352936568;314.159265358979 314.159265358979 314.159265358979;0.0797141621899262 2.2831725803905 0.714687245751717]  x4=[4.92919447329487 1717.64768099136 1720.51242220497;314.159265358979 314.159265358979 314.159265358979;-3.10619971926272 -0.858228555004222 -2.42671535526883]  x5=6.70710350311308e-07  V1=ones(3,3)  V2=ones(3,3)  I1=ones(3,3)  I2=ones(3,3)  nHarmo=1  Measurements=None  Decoupling=off  VsMag0=0  VrMag0=0  VsAngle0=0  VrAngle0=0  IsMag0=0  IrMag0=0  IsAngle0=0  IrAngle0=0
      settings: SourceProductBaseCode=PS
  Line 70 : spsDistributedParametersLineLib/Distributed Parameters Line  Phases=3  Length=0.50001  Frequency=50  Resistance=[0.646656091154803 0.0486237908083191 0.0486712220507153;0.0486237908083191 0.646561225344642 0.0486237934466192;0.0486712220507153 0.0486237934466192 0.646656091154803]  Inductance=[0.00282448912315926 0.00133270803418135 0.00132951476746136;0.00133270803418135 0.00282479813276775 0.00133799988507366;0.00132951476746136 0.00133799988507366 0.00282448912315926]  Capacitance=[7.89543174552926e-09 -1.85986777702161e-09 -1.7901190036642e-09;-1.85986777702161e-09 7.82540023894543e-09 -1.8957321828871e-09;-1.7901190036642e-09 -1.8957321828871e-09 7.91264394645417e-09]  x1=[115.996841356898 8377.57299190723 8377.59454867642;314.159265358979 314.159265358979 314.159265358979;0.8880395681714 -0.319530419879017 -1.8910200669477]  x2=[119.515985029828 7728.34046847707 7728.71589031762;314.159265358979 314.159265358979 314.159265358979;0.900500873844123 -0.330253962646824 -1.90171047174083]  x3=[4.14035625445154 1703.6220259809 1707.0118299354;314.159265358979 314.159265358979 314.159265358979;0.142593302100893 2.27639091979038 0.707748938472507]  x4=[3.99239849445041 1738.87991699736 1742.60073084927;314.159265358979 314.159265358979 314.159265358979;-3.03420701513013 -0.853085054128906 -2.42171737862123]  x5=2.3957842710327e-06  V1=ones(3,3)  V2=ones(3,3)  I1=ones(3,3)  I2=ones(3,3)  nHarmo=1  Measurements=None  Decoupling=off  VsMag0=0  VrMag0=0  VsAngle0=0  VrAngle0=0  IsMag0=0  IrMag0=0  IsAngle0=0  IrAngle0=0
      settings: SourceProductBaseCode=PS
  Line 71 : spsDistributedParametersLineLib/Distributed Parameters Line  Phases=3  Length=0.17  Frequency=50  Resistance=[0.646656091154803 0.0486237908083191 0.0486712220507153;0.0486237908083191 0.646561225344642 0.0486237934466192;0.0486712220507153 0.0486237934466192 0.646656091154803]  Inductance=[0.00282448912315926 0.00133270803418135 0.00132951476746136;0.00133270803418135 0.00282479813276775 0.00133799988507366;0.00132951476746136 0.00133799988507366 0.00282448912315926]  Capacitance=[7.89543174552926e-09 -1.85986777702161e-09 -1.7901190036642e-09;-1.85986777702161e-09 7.82540023894543e-09 -1.8957321828871e-09;-1.7901190036642e-09 -1.8957321828871e-09 7.91264394645417e-09]  x1=[115.996841356898 8377.57299190723 8377.59454867642;314.159265358979 314.159265358979 314.159265358979;0.888536327454891 -0.319135777254444 -1.89062504865129]  x2=[115.998529063803 8377.32656078335 8377.34861087559;314.159265358979 314.159265358979 314.159265358979;0.888541828518647 -0.319140505136676 -1.89062968060623]  x3=[0.105425727484544 19.6502394657352 19.8131762558927;314.159265358979 314.159265358979 314.159265358979;0.849806249448654 -0.271545176210544 -1.84344290424173]  x4=[0.0975625861376001 23.0222856189487 23.1864825859964;314.159265358979 314.159265358979 314.159265358979;0.930129133221467 -0.359944448357748 -1.93113178394843]  x5=8.14550361143895e-07  V1=ones(3,3)  V2=ones(3,3)  I1=ones(3,3)  I2=ones(3,3)  nHarmo=1  Measurements=None  Decoupling=off  VsMag0=0  VrMag0=0  VsAngle0=0  VrAngle0=0  IsMag0=0  IrMag0=0  IsAngle0=0  IrAngle0=0
      settings: SourceProductBaseCode=PS
  Line 72 : spsDistributedParametersLineLib/Distributed Parameters Line  Phases=3  Length=0.27999  Frequency=50  Resistance=[0.646656091154803 0.0486237908083191 0.0486712220507153;0.0486237908083191 0.646561225344642 0.0486237934466192;0.0486712220507153 0.0486237934466192 0.646656091154803]  Inductance=[0.00282448912315926 0.00133270803418135 0.00132951476746136;0.00133270803418135 0.00282479813276775 0.00133799988507366;0.00132951476746136 0.00133799988507366 0.00282448912315926]  Capacitance=[7.89543174552926e-09 -1.85986777702161e-09 -1.7901190036642e-09;-1.85986777702161e-09 7.82540023894543e-09 -1.8957321828871e-09;-1.7901190036642e-09 -1.8957321828871e-09 7.91264394645417e-09]  x1=[114.031669198193 8741.89960480062 8741.71991555675;314.159265358979 314.159265358979 314.159265358979;0.881048256462575 -0.313951062738499 -1.88545664682667]  x2=[115.996841356898 8377.57299190723 8377.59454867642;314.159265358979 314.159265358979 314.159265358979;0.888370761097535 -0.319267308851295 -1.89075670545691]  x3=[4.1455746277566 1705.09906766063 1708.48507591302;314.159265358979 314.159265358979 314.159265358979;0.142426938040057 2.27636096019249 0.70771593053669]  x4=[3.9996688004019 1742.41099617941 1746.14769883144;314.159265358979 314.159265358979 314.159265358979;-3.03315175503734 -0.852198024315638 -2.42083244378151]  x5=1.341564444804e-06  V1=ones(3,3)  V2=ones(3,3)  I1=ones(3,3)  I2=ones(3,3)  nHarmo=1  Measurements=None  Decoupling=off  VsMag0=0  VrMag0=0  VsAngle0=0  VrAngle0=0  IsMag0=0  IrMag0=0  IsAngle0=0  IrAngle0=0
      settings: SourceProductBaseCode=PS
  Line 73 : spsDistributedParametersLineLib/Distributed Parameters Line  Phases=3  Length=0.01  Frequency=50  Resistance=[0.646656091154803 0.0486237908083191 0.0486712220507153;0.0486237908083191 0.646561225344642 0.0486237934466192;0.0486712220507153 0.0486237934466192 0.646656091154803]  Inductance=[0.00282448912315926 0.00133270803418135 0.00132951476746136;0.00133270803418135 0.00282479813276775 0.00133799988507366;0.00132951476746136 0.00133799988507366 0.00282448912315926]  Capacitance=[7.89543174552926e-09 -1.85986777702161e-09 -1.7901190036642e-09;-1.85986777702161e-09 7.82540023894543e-09 -1.8957321828871e-09;-1.7901190036642e-09 -1.8957321828871e-09 7.91264394645417e-09]  x1=[113.961596700912 8754.91608914536 8754.72918567991;314.159265358979 314.159265358979 314.159265358979;0.881188474311274 -0.313446504254441 -1.88495232985911]  x2=[114.031669198193 8741.89960480062 8741.71991555675;314.159265358979 314.159265358979 314.159265358979;0.881454668507511 -0.31362819506113 -1.88513347180213]  x3=[4.14591470744199 1705.4211384376 1708.81019063931;314.159265358979 314.159265358979 314.159265358979;0.142819115160637 2.27667106374897 0.708026323229045]  x4=[4.00075627923751 1743.50539835299 1747.25263376271;314.159265358979 314.159265358979 314.159265358979;-3.03232145609305 -0.851542409845743 -2.42017622019573]  x5=4.79147271261115e-08  V1=ones(3,3)  V2=ones(3,3)  I1=ones(3,3)  I2=ones(3,3)  nHarmo=1  Measurements=None  Decoupling=off  VsMag0=0  VrMag0=0  VsAngle0=0  VrAngle0=0  IsMag0=0  IrMag0=0  IsAngle0=0  IrAngle0=0
      settings: SourceProductBaseCode=PS
  Line 74 : spsDistributedParametersLineLib/Distributed Parameters Line  Phases=3  Length=0.04  Frequency=50  Resistance=[0.646656091154803 0.0486237908083191 0.0486712220507153;0.0486237908083191 0.646561225344642 0.0486237934466192;0.0486712220507153 0.0486237934466192 0.646656091154803]  Inductance=[0.00282448912315926 0.00133270803418135 0.00132951476746136;0.00133270803418135 0.00282479813276775 0.00133799988507366;0.00132951476746136 0.00133799988507366 0.00282448912315926]  Capacitance=[7.89543174552926e-09 -1.85986777702161e-09 -1.7901190036642e-09;-1.85986777702161e-09 7.82540023894543e-09 -1.8957321828871e-09;-1.7901190036642e-09 -1.8957321828871e-09 7.91264394645417e-09]  x1=[113.681387453804 8806.98488276711 8806.76910503673;314.159265358979 314.159265358979 314.159265358979;0.880075258897803 -0.312760985589722 -1.88426902172254]  x2=[113.961596700912 8754.91608914536 8754.72918567991;314.159265358979 314.159265358979 314.159265358979;0.881143315744852 -0.313482379769538 -1.88498823952516]  x3=[4.14576825289747 1705.27749110482 1708.66517111353;314.159265358979 314.159265358979 314.159265358979;0.142714084111381 2.27658701499381 0.707942191892173]  x4=[4.00074411799732 1743.49162543123 1747.23872400763;314.159265358979 314.159265358979 314.159265358979;-3.03235136637686 -0.851566501173182 -2.42020033572968]  x5=1.91658908504446e-07  V1=ones(3,3)  V2=ones(3,3)  I1=ones(3,3)  I2=ones(3,3)  nHarmo=1  Measurements=None  Decoupling=off  VsMag0=0  VrMag0=0  VsAngle0=0  VrAngle0=0  IsMag0=0  IrMag0=0  IsAngle0=0  IrAngle0=0
      settings: SourceProductBaseCode=PS
  Line 8 : spsDistributedParametersLineLib/Distributed Parameters Line  Phases=3  Length=0.14997  Frequency=50  Resistance=[0.476003738225748 0.351747138225748 0.351747138225748;0.351747138225748 0.476003738225748 0.351747138225748;0.351747138225748 0.351747138225748 0.476003738225748]  Inductance=[0.000705954362986426 0.000459934243504405 0.000459934243504405;0.000459934243504405 0.000705954362986426 0.000459934243504405;0.000459934243504405 0.000459934243504405 0.000705954362986426]  Capacitance=[5.7561313269996e-07 -1.37543883484145e-07 -1.37543912800485e-07;-1.37543883484145e-07 5.75613027339387e-07 -1.37543875208088e-07;-1.37543912800485e-07 -1.37543875208088e-07 5.75613005057695e-07]  x1=[141.155515547976 1724.9901122593 1728.22364930304;314.159265358979 314.159265358979 314.159265358979;1.09231709391312 -0.771958676434234 -2.3408495793401]  x2=[141.155243232664 1712.67364194682 1715.88409144412;314.159265358979 314.159265358979 314.159265358979;1.09231535263046 -0.776393837517091 -2.34528474040656]  x3=[1.91310874048136 1619.78264452299 1622.81897453121;314.159265358979 314.159265358979 314.159265358979;1.09129052364173 2.36495794592835 0.796067040714612]  x4=[1.9224589479056 1804.8128375823 1808.19599698001;314.159265358979 314.159265358979 314.159265358979;1.09293653540389 -0.776394178752905 -2.34528508374587]  x5=1.27732009810033e-06  V1=ones(3,3)  V2=ones(3,3)  I1=ones(3,3)  I2=ones(3,3)  nHarmo=1  Measurements=None  Decoupling=off  VsMag0=0  VrMag0=0  VsAngle0=0  VrAngle0=0  IsMag0=0  IrMag0=0  IsAngle0=0  IrAngle0=0
      settings: SourceProductBaseCode=PS
  Line 9 : spsDistributedParametersLineLib/Distributed Parameters Line  Phases=3  Length=0.50001  Frequency=50  Resistance=[0.646656091154803 0.0486237908083191 0.0486712220507153;0.0486237908083191 0.646561225344642 0.0486237934466192;0.0486712220507153 0.0486237934466192 0.646656091154803]  Inductance=[0.00282448912315926 0.00133270803418135 0.00132951476746136;0.00133270803418135 0.00282479813276775 0.00133799988507366;0.00132951476746136 0.00133799988507366 0.00282448912315926]  Capacitance=[7.89543174552926e-09 -1.85986777702161e-09 -1.7901190036642e-09;-1.85986777702161e-09 7.82540023894543e-09 -1.8957321828871e-09;-1.7901190036642e-09 -1.8957321828871e-09 7.91264394645417e-09]  x1=[152.36017586446 2437.89117531741 2440.98179824564;314.159265358979 314.159265358979 314.159265358979;0.986478778428195 -0.642166502474468 -2.21226944400452]  x2=[156.941937925151 1872.28617161936 1875.3144168448;314.159265358979 314.159265358979 314.159265358979;0.993413033048069 -0.794094270612423 -2.36330510281402]  x3=[5.09935678304616 1708.0029446588 1710.76758951413;314.159265358979 314.159265358979 314.159265358979;0.0771565194109427 2.28213673898177 0.713650660601269]  x4=[4.93858001532251 1718.81092201543 1721.67640144465;314.159265358979 314.159265358979 314.159265358979;-3.10775431948524 -0.858499116228776 -2.42698593041487]  x5=2.3957842710327e-06  V1=ones(3,3)  V2=ones(3,3)  I1=ones(3,3)  I2=ones(3,3)  nHarmo=1  Measurements=None  Decoupling=off  VsMag0=0  VrMag0=0  VsAngle0=0  VrAngle0=0  IsMag0=0  IrMag0=0  IsAngle0=0  IrAngle0=0
      settings: SourceProductBaseCode=PS
  Line im1 : spsDistributedParametersLineLib/Distributed Parameters Line  Phases=3  Length=1e-10  Frequency=50  Resistance=[0.646656091154803 0.0486237908083191 0.0486712220507153;0.0486237908083191 0.646561225344642 0.0486237934466192;0.0486712220507153 0.0486237934466192 0.646656091154803]  Inductance=[0.00282448912315926 0.00133270803418135 0.00132951476746136;0.00133270803418135 0.00282479813276775 0.00133799988507366;0.00132951476746136 0.00133799988507366 0.00282448912315926]  Capacitance=[7.89543174552926e-09 -1.85986777702161e-09 -1.7901190036642e-09;-1.85986777702161e-09 7.82540023894543e-09 -1.8957321828871e-09;-1.7901190036642e-09 -1.8957321828871e-09 7.91264394645417e-09]  x1=[156.969311652178 1871.26228409431 1874.29035744918;314.159265358979 314.159265358979 314.159265358979;0.994096285113969 -0.793886332727418 -2.36309431363867]  x2=[156.969311652266 1871.26228409423 1874.29035744908;314.159265358979 314.159265358979 314.159265358979;0.994096285114001 -0.793886332727482 -2.36309431363867]  x3=[0.543972443374269 3.10625052498748 3.87895543149896;314.159265358979 314.159265358979 314.159265358979;0.113271303177305 -1.00963093185153 -2.14546198539272]  x4=[0.423712714032155 6.52129418743106 5.88238382407158;314.159265358979 314.159265358979 314.159265358979;2.73513311644566 -0.691934659459349 -2.50607669012292]  x5=4.79147271261115e-16  V1=ones(3,3)  V2=ones(3,3)  I1=ones(3,3)  I2=ones(3,3)  nHarmo=1  Measurements=None  Decoupling=off  VsMag0=0  VrMag0=0  VsAngle0=0  VrAngle0=0  IsMag0=0  IrMag0=0  IsAngle0=0  IrAngle0=0
      settings: SourceProductBaseCode=PS
  Line im2 : spsDistributedParametersLineLib/Distributed Parameters Line  Phases=3  Length=1e-10  Frequency=50  Resistance=[0.646656091154803 0.0486237908083191 0.0486712220507153;0.0486237908083191 0.646561225344642 0.0486237934466192;0.0486712220507153 0.0486237934466192 0.646656091154803]  Inductance=[0.00282448912315926 0.00133270803418135 0.00132951476746136;0.00133270803418135 0.00282479813276775 0.00133799988507366;0.00132951476746136 0.00133799988507366 0.00282448912315926]  Capacitance=[7.89543174552926e-09 -1.85986777702161e-09 -1.7901190036642e-09;-1.85986777702161e-09 7.82540023894543e-09 -1.8957321828871e-09;-1.7901190036642e-09 -1.8957321828871e-09 7.91264394645417e-09]  x1=[149.339597082436 2831.70975810682 2834.63941733118;314.159265358979 314.159265358979 314.159265358979;0.982421456467797 -0.575463928961506 -2.14591380818243]  x2=[149.339597083058 2831.70975798566 2834.63941721022;314.159265358979 314.159265358979 314.159265358979;0.982421456470137 -0.575463928978772 -2.14591380819946]  x3=[3.91041417034116 1711.18102156419 1710.17620067071;314.159265358979 314.159265358979 314.159265358979;0.352106248691822 2.28239142198924 0.711222310896528]  x4=[3.70310989055191 1725.01815479729 1724.13412283573;314.159265358979 314.159265358979 314.159265358979;-2.83379174942435 -0.85686129574806 -2.42800212789897]  x5=4.79147271261115e-16  V1=ones(3,3)  V2=ones(3,3)  I1=ones(3,3)  I2=ones(3,3)  nHarmo=1  Measurements=None  Decoupling=off  VsMag0=0  VrMag0=0  VsAngle0=0  VrAngle0=0  IsMag0=0  IrMag0=0  IsAngle0=0  IrAngle0=0
      settings: SourceProductBaseCode=PS
  Line im3 : spsDistributedParametersLineLib/Distributed Parameters Line  Phases=3  Length=1e-10  Frequency=50  Resistance=[0.646656091154803 0.0486237908083191 0.0486712220507153;0.0486237908083191 0.646561225344642 0.0486237934466192;0.0486712220507153 0.0486237934466192 0.646656091154803]  Inductance=[0.00282448912315926 0.00133270803418135 0.00132951476746136;0.00133270803418135 0.00282479813276775 0.00133799988507366;0.00132951476746136 0.00133799988507366 0.00282448912315926]  Capacitance=[7.89543174552926e-09 -1.85986777702161e-09 -1.7901190036642e-09;-1.85986777702161e-09 7.82540023894543e-09 -1.8957321828871e-09;-1.7901190036642e-09 -1.8957321828871e-09 7.91264394645417e-09]  x1=[130.220285493139 5778.64498281735 5780.03432490305;314.159265358979 314.159265358979 314.159265358979;0.934711016394114 -0.37648036457609 -1.9477818183032]  x2=[130.220285493845 5778.64498268911 5780.03432477456;314.159265358979 314.159265358979 314.159265358979;0.93471101639637 -0.376480364580211 -1.94778181830738]  x3=[4.16037392595237 1702.19836362722 1710.87881789621;314.159265358979 314.159265358979 314.159265358979;0.182966565906696 2.27860934609777 0.712845061125574]  x4=[4.0037466046743 1728.25843180984 1737.21109322521;314.159265358979 314.159265358979 314.159265358979;-2.99699627598989 -0.855028901192277 -2.42085771230208]  x5=4.79147271261115e-16  V1=ones(3,3)  V2=ones(3,3)  I1=ones(3,3)  I2=ones(3,3)  nHarmo=1  Measurements=None  Decoupling=off  VsMag0=0  VrMag0=0  VsAngle0=0  VrAngle0=0  IsMag0=0  IrMag0=0  IsAngle0=0  IrAngle0=0
      settings: SourceProductBaseCode=PS
  Load {1,6,8041,8173} (4 alike) : spsThreePhaseSeriesRLCLoadLib/Three-Phase Series RLC Load  LConnTagsString=A|B|C  Configuration=Delta  NominalVoltage=11000  Vabc=[1e3 1e3 1e3]  Vabcp=[1e3 1e3 1e3]  NominalFrequency=50  UnbalancedPower=off  ActivePower=28052.64  InductivePower=13586.514  CapacitivePower=0  Pabc=[10e3 9e3 11e3]  QLabc=[100 90 110]  QCabc=[100 90 110]  Pabcp=[10e3 9e3 11e3]  QLabcp=[100 90 110]  QCabcp=[100 90 110]  Measurements=None  LoadType=constant Z
  Load {5,10,8293,8733} (4 alike) : spsThreePhaseSeriesRLCLoadLib/Three-Phase Series RLC Load  LConnTagsString=A|B|C  Configuration=Delta  NominalVoltage=11000  Vabc=[1e3 1e3 1e3]  Vabcp=[1e3 1e3 1e3]  NominalFrequency=50  UnbalancedPower=off  ActivePower=7013.16  InductivePower=3396.628  CapacitivePower=0  Pabc=[10e3 9e3 11e3]  QLabc=[100 90 110]  QCabc=[100 90 110]  Pabcp=[10e3 9e3 11e3]  QLabcp=[100 90 110]  QCabcp=[100 90 110]  Measurements=None  LoadType=constant Z
  Load {2..3,7..8,8287,8485} (6 alike) : spsThreePhaseSeriesRLCLoadLib/Three-Phase Series RLC Load  LConnTagsString=A|B|C  Configuration=Delta  NominalVoltage=11000  Vabc=[1e3 1e3 1e3]  Vabcp=[1e3 1e3 1e3]  NominalFrequency=50  UnbalancedPower=off  ActivePower=35065.8  InductivePower=16983.142  CapacitivePower=0  Pabc=[10e3 9e3 11e3]  QLabc=[100 90 110]  QCabc=[100 90 110]  Pabcp=[10e3 9e3 11e3]  QLabcp=[100 90 110]  QCabcp=[100 90 110]  Measurements=None  LoadType=constant Z
  Load 4 : spsThreePhaseSeriesRLCLoadLib/Three-Phase Series RLC Load  LConnTagsString=A|B|C  Configuration=Delta  NominalVoltage=11000  Vabc=[1e3 1e3 1e3]  Vabcp=[1e3 1e3 1e3]  NominalFrequency=50  UnbalancedPower=off  ActivePower=280.526  InductivePower=135.865  CapacitivePower=0  Pabc=[10e3 9e3 11e3]  QLabc=[100 90 110]  QCabc=[100 90 110]  Pabcp=[10e3 9e3 11e3]  QLabcp=[100 90 110]  QCabcp=[100 90 110]  Measurements=None  LoadType=constant Z
  Load 8424 : spsThreePhaseSeriesRLCLoadLib/Three-Phase Series RLC Load  LConnTagsString=A|B|C  Configuration=Delta  NominalVoltage=11000  Vabc=[1e3 1e3 1e3]  Vabcp=[1e3 1e3 1e3]  NominalFrequency=50  UnbalancedPower=off  ActivePower=11221.056  InductivePower=5434.605  CapacitivePower=0  Pabc=[10e3 9e3 11e3]  QLabc=[100 90 110]  QCabc=[100 90 110]  Pabcp=[10e3 9e3 11e3]  QLabcp=[100 90 110]  QCabcp=[100 90 110]  Measurements=None  LoadType=constant Z
  Load 8551 : spsThreePhaseSeriesRLCLoadLib/Three-Phase Series RLC Load  LConnTagsString=A|B|C  Configuration=Delta  NominalVoltage=11000  Vabc=[1e3 1e3 1e3]  Vabcp=[1e3 1e3 1e3]  NominalFrequency=50  UnbalancedPower=off  ActivePower=11221.056  InductivePower=5434.605  CapacitivePower=0  Pabc=[10e3 9e3 11e3]  QLabc=[100 90 110]  QCabc=[100 90 110]  Pabcp=[10e3 9e3 11e3]  QLabcp=[100 90 110]  QCabcp=[100 90 110]  Measurements=None  LoadType=constant Z
  Load 8605 : spsThreePhaseSeriesRLCLoadLib/Three-Phase Series RLC Load  LConnTagsString=A|B|C  Configuration=Delta  NominalVoltage=11000  Vabc=[1e3 1e3 1e3]  Vabcp=[1e3 1e3 1e3]  NominalFrequency=50  UnbalancedPower=off  ActivePower=280.526  InductivePower=135.865  CapacitivePower=0  Pabc=[10e3 9e3 11e3]  QLabc=[100 90 110]  QCabc=[100 90 110]  Pabcp=[10e3 9e3 11e3]  QLabcp=[100 90 110]  QCabcp=[100 90 110]  Measurements=None  LoadType=constant Z
  Load 8737 : spsThreePhaseSeriesRLCLoadLib/Three-Phase Series RLC Load  LConnTagsString=A|B|C  Configuration=Delta  NominalVoltage=11000  Vabc=[1e3 1e3 1e3]  Vabcp=[1e3 1e3 1e3]  NominalFrequency=50  UnbalancedPower=off  ActivePower=17532.9  InductivePower=8491.571  CapacitivePower=0  Pabc=[10e3 9e3 11e3]  QLabc=[100 90 110]  QCabc=[100 90 110]  Pabcp=[10e3 9e3 11e3]  QLabcp=[100 90 110]  QCabcp=[100 90 110]  Measurements=None  LoadType=constant Z
  Load 9 : spsThreePhaseSeriesRLCLoadLib/Three-Phase Series RLC Load  LConnTagsString=A|B|C  Configuration=Delta  NominalVoltage=11000  Vabc=[1e3 1e3 1e3]  Vabcp=[1e3 1e3 1e3]  NominalFrequency=50  UnbalancedPower=off  ActivePower=280.526  InductivePower=135.865  CapacitivePower=0  Pabc=[10e3 9e3 11e3]  QLabc=[100 90 110]  QCabc=[100 90 110]  Pabcp=[10e3 9e3 11e3]  QLabcp=[100 90 110]  QCabcp=[100 90 110]  Measurements=None  LoadType=constant Z
  R{1..3,5} (4 alike) : spsThreePhaseVIMeasurementLib/Three-Phase V-I Measurement  VoltageMeasurement=phase-to-ground  SetLabelV=off  LabelV=Vabc  Vpu=off  VpuLL=off  CurrentMeasurement=yes  SetLabelI=off  LabelI=Iabc  Ipu=off  Pbase=100e6  Vbase=500e3  OutputType=Complex  PhasorSimulation=on  PSBequivalent=0
  Scope R{1..3,5} (4 alike) : Scope  NumInputPorts=2
  Source PC1_TT2 : spsThreePhaseSourceLib/Three-Phase Source  InternalConnection=Yn  VoltagePhases=off  Voltage=10000  PhaseAngle=0  Voltage_phases=[25e3 25e3 25e3]/sqrt(3)  PhaseAngles_phases=[0 -120 +120]  Frequency=50  NonIdealSource=on  SpecifyImpedance=off  Resistance=0.14  Inductance=0.0031831  ShortCircuitLevel=100e6  BaseVoltage=25e3  XRratio=7  BusType=swing  Pref=10e3  Qref=0  Prefabc=[10e3, 10e3, 10e3]  Qrefabc=[0, 0, 0]  Qmin=-inf  Qmax=inf
  Source Zn : spsSeriesRLCBranchLib/Series RLC Branch  LConnTagsString=__new0  RConnTagsString=__new0  BranchType=RL  Resistance=0.001  Inductance=3.1831e-06  SetiL0=off  InitialCurrent=0  Capacitance=0  Setx0=off  InitialVoltage=0  Measurements=None
  powergui : spspowerguiLib/powergui  Priority=1  SimulationMode=Phasor  SampleTime=50e-6  frequency=50  Iterations=50  frequencyindice=50  Pbase=100e6  ErrMax=1e-4  UnitsV=kV  UnitsW=MW  buscounter=0  FunctionMessages=off  echomessages=off  EnableUseOfTLC=off  CurrentSourceSwitches=off  DisableSnubberDevices=off  DisableRonSwitches=off  DisableVfSwitches=off  DisplayEquations=off  AutomaticDiscreteSolvers=off  SolverType=Tustin/Backward Euler (TBE)  Interpol=off  ExternalGateDelay=off  methode=off  Ts=10  x0status=blocks  SPID=off  SwTol=0  HookPort=off  NonlinearTolerance=1e-4  nMaxIteration=100  ContinueOnMaxIteration=off  RestoreLinks=warning  ResistiveCurrentMeasurement=off  Frange=[0:2:500]  Ylog=off  Xlog=on  ShowGrid=off  save=off  variable=ZData  structure=0  ZoomFFT=off  StartTime=0.0  cycles=1  DisplayStyle=1  fundamental=60  FreqAxis=off  MaxFrequency=1000  frequencyindicesteady=1  RmsSteady=1  display=off
  wires:
  R5/2 -> Scope R5/2
  R2/1 -> Scope R2/1
  R5/1 -> Scope R5/1
  R2/2 -> Scope R2/2
  R3/2 -> Scope R3/2
  R3/1 -> Scope R3/1
  R1/1 -> Scope R1/1
  R1/2 -> Scope R1/2
  connections:
  Source Zn/RConn1 -- Source PC1_TT2/LConn1
  Source Zn/LConn1 -- Ground/LConn1
  Line 66/LConn1 -- Line 65/LConn1 -- Line 67/RConn1
  Line 66/LConn2 -- Line 65/LConn2 -- Line 67/RConn2
  Line 66/LConn3 -- Line 65/LConn3 -- Line 67/RConn3
  Line 2/LConn1 -- Line 1/LConn1 -- Line 3/RConn1
  Line 2/LConn2 -- Line 1/LConn2 -- Line 3/RConn2
  Line 2/LConn3 -- Line 1/LConn3 -- Line 3/RConn3
  Line 19/LConn1 -- Line 14/LConn1 -- Line 20/RConn1
  Line 19/LConn2 -- Line 14/LConn2 -- Line 20/RConn2
  Line 19/LConn3 -- Line 14/LConn3 -- Line 20/RConn3
  Line 68/RConn1 -- Line 69/LConn1
  Line 68/RConn2 -- Line 69/LConn2
  Line 68/RConn3 -- Line 69/LConn3
  Line 71/LConn1 -- Line 70/LConn1 -- Line 72/RConn1
  Line 71/LConn2 -- Line 70/LConn2 -- Line 72/RConn2
  Line 71/LConn3 -- Line 70/LConn3 -- Line 72/RConn3
  Load 8733/LConn1 -- Line 63/RConn1
  Load 8733/LConn2 -- Line 63/RConn2
  Load 8733/LConn3 -- Line 63/RConn3
  Source PC1_TT2/RConn1 -- R2/LConn1
  Source PC1_TT2/RConn2 -- R2/LConn2
  Source PC1_TT2/RConn3 -- R2/LConn3
  Line 18/LConn1 -- Line im3/RConn1
  Line 18/LConn2 -- Line im3/RConn2
  Line 18/LConn3 -- Line im3/RConn3
  Line im3/LConn1 -- R5/RConn1
  Line im3/LConn2 -- R5/RConn2
  Line im3/LConn3 -- R5/RConn3
  Load 3/LConn1 -- Line 3/LConn1 -- Line 4/RConn1
  Load 3/LConn2 -- Line 3/LConn2 -- Line 4/RConn2
  Load 3/LConn3 -- Line 3/LConn3 -- Line 4/RConn3
  Load 8485/LConn1 -- Line 64/LConn1 -- Line 65/RConn1
  Load 8485/LConn2 -- Line 64/LConn2 -- Line 65/RConn2
  Load 8485/LConn3 -- Line 64/LConn3 -- Line 65/RConn3
  Line 17/LConn1 -- Line 18/RConn1
  Line 17/LConn2 -- Line 18/RConn2
  Line 17/LConn3 -- Line 18/RConn3
  Line 63/LConn1 -- Line 62/LConn1 -- Line 64/RConn1
  Line 63/LConn2 -- Line 62/LConn2 -- Line 64/RConn2
  Line 63/LConn3 -- Line 62/LConn3 -- Line 64/RConn3
  Line 15/RConn1 -- Load 6/LConn1
  Line 15/RConn2 -- Load 6/LConn2
  Line 15/RConn3 -- Load 6/LConn3
  Load 8/LConn1 -- Line 20/LConn1 -- Line 21/RConn1
  Load 8/LConn2 -- Line 20/LConn2 -- Line 21/RConn2
  Load 8/LConn3 -- Line 20/LConn3 -- Line 21/RConn3
  Line 56/LConn1 -- Line 55/LConn1 -- Line 54/RConn1
  Line 56/LConn2 -- Line 55/LConn2 -- Line 54/RConn2
  Line 56/LConn3 -- Line 55/LConn3 -- Line 54/RConn3
  Line 5/RConn1 -- Load 4/LConn1
  Line 5/RConn2 -- Load 4/LConn2
  Line 5/RConn3 -- Load 4/LConn3
  Line 16/LConn1 -- Line 17/RConn1
  Line 16/LConn2 -- Line 17/RConn2
  Line 16/LConn3 -- Line 17/RConn3
  Line 58/RConn1 -- Load 8551/LConn1
  Line 58/RConn2 -- Load 8551/LConn2
  Line 58/RConn3 -- Load 8551/LConn3
  Line 7/RConn1 -- Line 8/LConn1
  Line 7/RConn2 -- Line 8/LConn2
  Line 7/RConn3 -- Line 8/LConn3
  Line 58/LConn1 -- Line 57/LConn1 -- Line 56/RConn1
  Line 58/LConn2 -- Line 57/LConn2 -- Line 56/RConn2
  Line 58/LConn3 -- Line 57/LConn3 -- Line 56/RConn3
  Line 25/RConn1 -- Load 7/LConn1
  Line 25/RConn2 -- Load 7/LConn2
  Line 25/RConn3 -- Load 7/LConn3
  Line 11/LConn1 -- Line 12/RConn1
  Line 11/LConn2 -- Line 12/RConn2
  Line 11/LConn3 -- Line 12/RConn3
  Line 54/LConn1 -- Line 53/LConn1 -- Line 59/RConn1
  Line 54/LConn2 -- Line 53/LConn2 -- Line 59/RConn2
  Line 54/LConn3 -- Line 53/LConn3 -- Line 59/RConn3
  Line 55/RConn1 -- Load 8424/LConn1
  Line 55/RConn2 -- Load 8424/LConn2
  Line 55/RConn3 -- Load 8424/LConn3
  Line im1/LConn1 -- R3/RConn1
  Line im1/LConn2 -- R3/RConn2
  Line im1/LConn3 -- R3/RConn3
  Line 24/RConn1 -- Line 25/LConn1
  Line 24/RConn2 -- Line 25/LConn2
  Line 24/RConn3 -- Line 25/LConn3
  Line 22/LConn1 -- Line 21/LConn1 -- Line 23/RConn1
  Line 22/LConn2 -- Line 21/LConn2 -- Line 23/RConn2
  Line 22/LConn3 -- Line 21/LConn3 -- Line 23/RConn3
  Line 10/RConn1 -- Load 1/LConn1
  Line 10/RConn2 -- Load 1/LConn2
  Line 10/RConn3 -- Load 1/LConn3
  Line 7/LConn1 -- Line 6/LConn1 -- Line 9/RConn1
  Line 7/LConn2 -- Line 6/LConn2 -- Line 9/RConn2
  Line 7/LConn3 -- Line 6/LConn3 -- Line 9/RConn3
  Line 74/LConn1 -- R2/RConn1
  Line 74/LConn2 -- R2/RConn2
  Line 74/LConn3 -- R2/RConn3
  Line 24/LConn1 -- Line 23/LConn1 -- Line 26/RConn1
  Line 24/LConn2 -- Line 23/LConn2 -- Line 26/RConn2
  Line 24/LConn3 -- Line 23/LConn3 -- Line 26/RConn3
  Load 10/LConn1 -- Line 19/RConn1
  Load 10/LConn2 -- Line 19/RConn2
  Load 10/LConn3 -- Line 19/RConn3
  Line im2/RConn1 -- Line 13/LConn1
  Line im2/RConn2 -- Line 13/LConn2
  Line im2/RConn3 -- Line 13/LConn3
  Line 22/RConn1 -- Load 9/LConn1
  Line 22/RConn2 -- Load 9/LConn2
  Line 22/RConn3 -- Load 9/LConn3
  Line 69/RConn1 -- Load 8287/LConn1
  Line 69/RConn2 -- Load 8287/LConn2
  Line 69/RConn3 -- Load 8287/LConn3
  Line 52/LConn1 -- Line 51/LConn1 -- Line 53/RConn1
  Line 52/LConn2 -- Line 51/LConn2 -- Line 53/RConn2
  Line 52/LConn3 -- Line 51/LConn3 -- Line 53/RConn3
  Line 68/LConn1 -- Line 67/LConn1 -- Line 70/RConn1
  Line 68/LConn2 -- Line 67/LConn2 -- Line 70/RConn2
  Line 68/LConn3 -- Line 67/LConn3 -- Line 70/RConn3
  Line 57/RConn1 -- Load 8293/LConn1
  Line 57/RConn2 -- Load 8293/LConn2
  Line 57/RConn3 -- Load 8293/LConn3
  Load 8737/LConn1 -- Line 52/RConn1
  Load 8737/LConn2 -- Line 52/RConn2
  Load 8737/LConn3 -- Line 52/RConn3
  Line 66/RConn1 -- Load 8605/LConn1
  Line 66/RConn2 -- Load 8605/LConn2
  Line 66/RConn3 -- Load 8605/LConn3
  Line im2/LConn1 -- R1/RConn1
  Line im2/LConn2 -- R1/RConn2
  Line im2/LConn3 -- R1/RConn3
  Line 62/RConn1 -- R5/LConn1
  Line 62/RConn2 -- R5/LConn2
  Line 62/RConn3 -- R5/LConn3
  Line 5/LConn1 -- Line 4/LConn1 -- Line 6/RConn1
  Line 5/LConn2 -- Line 4/LConn2 -- Line 6/RConn2
  Line 5/LConn3 -- Line 4/LConn3 -- Line 6/RConn3
  Line 49/LConn1 -- Line 48/LConn1 -- Line 47/RConn1
  Line 49/LConn2 -- Line 48/LConn2 -- Line 47/RConn2
  Line 49/LConn3 -- Line 48/LConn3 -- Line 47/RConn3
  Line 14/RConn1 -- R1/LConn1
  Line 14/RConn2 -- R1/LConn2
  Line 14/RConn3 -- R1/LConn3
  Line 71/RConn1 -- Load 8041/LConn1
  Line 71/RConn2 -- Load 8041/LConn2
  Line 71/RConn3 -- Load 8041/LConn3
  Line 60/RConn1 -- Line 61/LConn1
  Line 60/RConn2 -- Line 61/LConn2
  Line 60/RConn3 -- Line 61/LConn3
  Line 15/LConn1 -- Line 26/LConn1 -- Line 16/RConn1
  Line 15/LConn2 -- Line 26/LConn2 -- Line 16/RConn2
  Line 15/LConn3 -- Line 26/LConn3 -- Line 16/RConn3
  Line 73/LConn1 -- Line 74/RConn1
  Line 73/LConn2 -- Line 74/RConn2
  Line 73/LConn3 -- Line 74/RConn3
  Line 72/LConn1 -- Line 73/RConn1
  Line 72/LConn2 -- Line 73/RConn2
  Line 72/LConn3 -- Line 73/RConn3
  Line 12/LConn1 -- Line 13/RConn1
  Line 12/LConn2 -- Line 13/RConn2
  Line 12/LConn3 -- Line 13/RConn3
  Line 1/RConn1 -- R3/LConn1
  Line 1/RConn2 -- R3/LConn2
  Line 1/RConn3 -- R3/LConn3
  Line 44/LConn1 -- Line 45/RConn1
  Line 44/LConn2 -- Line 45/RConn2
  Line 44/LConn3 -- Line 45/RConn3
  Line 45/LConn1 -- Line 46/LConn1 -- Load 8173/LConn1 -- Line 50/RConn1
  Line 45/LConn2 -- Line 46/LConn2 -- Load 8173/LConn2 -- Line 50/RConn2
  Line 45/LConn3 -- Line 46/LConn3 -- Load 8173/LConn3 -- Line 50/RConn3
  Line 60/LConn1 -- Line 59/LConn1 -- Line im1/RConn1
  Line 60/LConn2 -- Line 59/LConn2 -- Line im1/RConn2
  Line 60/LConn3 -- Line 59/LConn3 -- Line im1/RConn3
  Line 10/LConn1 -- Line 9/LConn1 -- Line 11/RConn1
  Line 10/LConn2 -- Line 9/LConn2 -- Line 11/RConn2
  Line 10/LConn3 -- Line 9/LConn3 -- Line 11/RConn3
  Line 46/RConn1 -- Line 47/LConn1
  Line 46/RConn2 -- Line 47/LConn2
  Line 46/RConn3 -- Line 47/LConn3
  Line 51/RConn1 -- Line 50/LConn1
  Line 51/RConn2 -- Line 50/LConn2
  Line 51/RConn3 -- Line 50/LConn3
  Load 5/LConn1 -- Line 2/RConn1
  Load 5/LConn2 -- Line 2/RConn2
  Load 5/LConn3 -- Line 2/RConn3
  Line 8/RConn1 -- Load 2/LConn1
  Line 8/RConn2 -- Load 2/LConn2
  Line 8/RConn3 -- Load 2/LConn3
